simulink model "Australian14gen_inertia"  (R2017b)
settings: Solver=ode23tb  StartTime=0.0  StopTime=50  FixedStep=1e-3  RelTol=1e-3  AbsTol=1e-3  EnableMultiTasking=on
PreLoadFcn:
  | dataaustralian14gen
values from neighbouring files (symbols this model uses):
  alpha = -sys.follin.opt.alpha*1e8    [main_following.m]    (also in optimgains.mat = [-2447350365.29 -12566370614.4 -12566370614.4 -11730281347.7)
  bus_v = [ 101	15 ... (first row only)    [dataaustralian14gen.m]
  comp = [ 1	211	0	0 ... (first row only)    [dataaustralian14gen.m]
  dist = sys.follin.dist    [main_following.m]    (also in main_forming.m = sys.formin.dist)
  Exc = [ 101	0	 200	0.1	    13.25  2.5	 0	0       0       0       0       0 ... (first row only)    [dataaustralian14gen.m]
  FH = 13    [dataaustralian14gen.m]
  FI = 1    [dataaustralian14gen.m]
  FL = .1    (= 0.1)    [dataaustralian14gen.m]
  G_data = [ 101	333.3	15	3.6	0.14	1.1	0.65	0.25	8.5     0.25	0.05	0       0       0.25	0.2 	0 ... (first row only)    [dataaustralian14gen.m]
  KH = 120    [dataaustralian14gen.m]
  KI = 10    [dataaustralian14gen.m]
  KL = 10    [dataaustralian14gen.m]
  Kvsc = [-4.89904313526 -21.043852985 -7.4754770322 -20.8245159401 -7.65455531538 -20.65157337 -7.20128124012 -20.8334958357 -6.74777960012 -20.6206111903 -7.78863485578 -20.7555924998 ... (30 elements, 2x15)]    [optimgains.mat]
  line = [ 102	217	0.0084	0.0667	0.817	330	1 ... (first row only)    [dataaustralian14gen.m]
  load_mag = load_case4    [dataaustralian14gen.m]
  p = p_case4    [dataaustralian14gen.m]
  Pinit = zeros(15,1)    [dataaustralian14gen.m]
  PLL_Ki = 2/500    (= 0.004)    [dataaustralian14gen.m]
  PLL_Kp = 2/500    (= 0.004)    [dataaustralian14gen.m]
  PSSMODEL = 1    [dataaustralian14gen.m]
  trans = [ 1	101	102	15	330	333.3	12	12 ... (first row only)    [dataaustralian14gen.m]
undefined symbols (not defined in the file or in its folder): D1, Delta, sys, thetavsc0, Vbase
libraries: powerlib x388, Library x60, powerlib_meascontrol x15, sps_avr x10, powerlib_extras x4
(part 1 of 5)
Description:
  | SimPowerSystem model of the Simplified 14-Generator model
  | of the SE Australian Power System developed by Mike Gibbard & David Vowles,
  | School of Electrical & Electronic Engineering, The university of Adelaide, south australia)
  | 
  | SimPowerSystems model and validations by Ali Moeini and Innocent Kamwa,
  | IREQ, Hydro-Québec, Canada
settings Model: Creator=IREQ  LastModifiedBy=dominic
settings DataIOCC: LimitDataPoints=on  SaveFormat=Array
settings OptimizationCC: ExpressionDepthLimit=2147483647  LifeSpan=inf
settings DebuggingCC: UnderspecifiedInitializationDetection=Classic  MergeDetectMultiDrivingBlocksExec=none  IgnoredZcDiagnostic=none  SolverPrmCheckMsg=warning  UnconnectedInputMsg=none  UnconnectedOutputMsg=none  UnconnectedLineMsg=none  StateNameClashWarn=warning  SFUnexpectedBacktrackingDiag=warning  SFNoUnconditionalDefaultTransitionDiag=warning  SFExecutionAtInitializationDiag=none
settings HardwareCC: ProdBitPerPointer=32  ProdBitPerSizeT=32  ProdBitPerPtrDiffT=32  ProdLargestAtomicFloat=None  ProdIntDivRoundTo=Undefined  ProdEndianess=Unspecified  ProdWordSize=32  ProdHWDeviceType=32-bit Generic
settings ModelReferenceCC: PropagateSignalLabelsOutOfModel=off
settings CodeAppCC: StateflowObjectComments=on
settings GRTTargetCC: TargetLangStandard=C89/C90 (ANSI)  GeneratePreprocessorConditionals=Disable all
settings ConfigComp: CovMetricSettings=dw  CovHtmlReporting=on  CovSaveCumulativeToWorkspaceVar=on  CovSaveSingleToWorkspaceVar=on  CovExternalEMLEnable=off  CovSFcnEnable=off
settings SimscapeCC: SimscapeNormalizeSystem=off

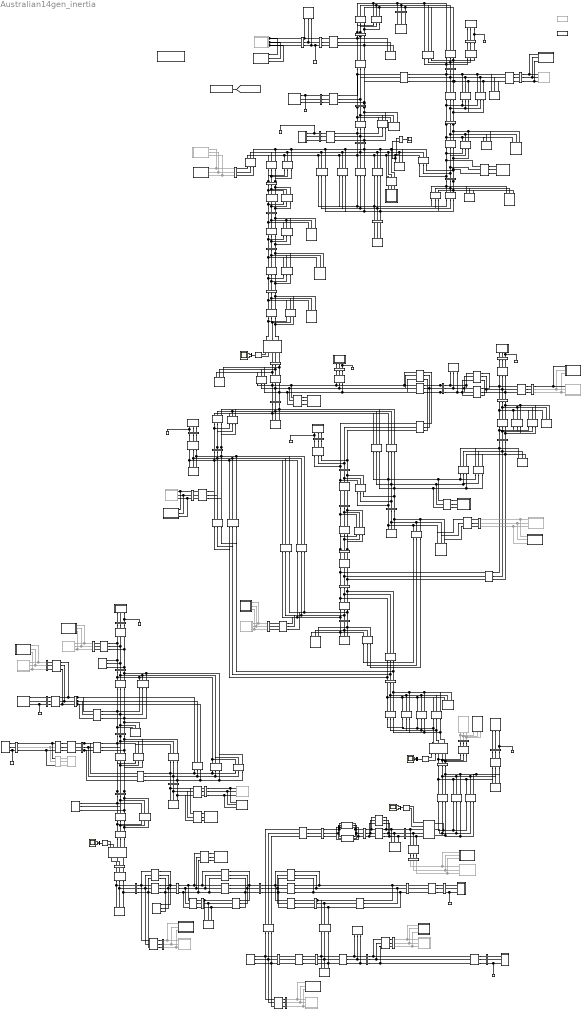
== system Australian14gen_inertia ==
  1 : powerlib/Elements/Three-Phase Series RLC Branch  LConnTagsString=A|B|C  RConnTagsString=A|B|C  BranchType=C  Resistance=0  Inductance=0  Capacitance=1/(0.0337)/(2*pi*50)*(330^2/100)  Measurements=None
  2 : powerlib/Elements/Three-Phase Series RLC Branch  LConnTagsString=A|B|C  RConnTagsString=A|B|C  BranchType=C  Resistance=0  Inductance=0  Capacitance=1/(0.0337)/(2*pi*50)*(330^2/100)  Measurements=None
  3-Phase Active & Reactive Power (Phasor Type){1..4} (4 alike) : powerlib_extras/Phasor Library/3-Phase Active & Reactive Power (Phasor Type)
  3-Phase Dynamic Load3 : powerlib/Elements/Three-Phase Dynamic Load  NominalVoltage=[ 15e3 50 ]  ActiveReactivePowers=[-5.4e+08 -4.56e+06]  PositiveSequence=[0.999196 -2.87767]  ExternalControl=off  NpNq="[0  0]"  TimeConstants=[0 0 0 0]  MinimumVoltage=0.01  Tfilter=1e-1  LoadFlowParameters=[4 50000000 0 0 25000000]
      settings: SourceProductName=Simscape Power Systems  SourceProductBaseCode=PS
  3-Phase Dynamic Load4 : powerlib/Elements/Three-Phase Dynamic Load  NominalVoltage=[ 15e3 50 ]  ActiveReactivePowers=[-1100 -2.11758e-14]  PositiveSequence=[1.08335 6.60259]  ExternalControl=off  NpNq="[0  0]"  TimeConstants=[0 0 0 0]  MinimumVoltage=0.01  Tfilter=1e-1  LoadFlowParameters=[4 50000000 0 0 25000000]
      settings: SourceProductName=Simscape Power Systems  SourceProductBaseCode=PS
  B101 : powerlib/Measurements/Three-Phase V-I Measurement  VoltageMeasurement=phase-to-phase  SetLabelV=on  LabelV=Vabc_B101  Vpu=off  VpuLL=off  CurrentMeasurement=no  SetLabelI=on  LabelI=Iabc_B101  Ipu=off  Pbase=100e6  Vbase=bus_v(1,2)*e3  OutputType=Complex  PhasorSimulation=on  PSBequivalent=0
  B102 : powerlib/Measurements/Three-Phase V-I Measurement  VoltageMeasurement=phase-to-ground  SetLabelV=on  LabelV=Vabc_B102  Vpu=off  VpuLL=off  CurrentMeasurement=yes  SetLabelI=on  LabelI=Iabc_B102  Ipu=off  Pbase=100e6  Vbase=bus_v(2,2)*e3  OutputType=Complex  PhasorSimulation=on  PSBequivalent=0
  B102_vi : powerlib/Measurements/Three-Phase V-I Measurement  VoltageMeasurement=phase-to-phase  SetLabelV=on  LabelV=Vabc_B102_vi  Vpu=off  VpuLL=off  CurrentMeasurement=no  SetLabelI=on  LabelI=Iabc_B101  Ipu=off  Pbase=100e6  Vbase=bus_v(1,2)*e3  OutputType=Complex  PhasorSimulation=on  PSBequivalent=0
  B201 : powerlib/Measurements/Three-Phase V-I Measurement  VoltageMeasurement=phase-to-phase  SetLabelV=on  LabelV=Vabc_B201  Vpu=off  VpuLL=off  CurrentMeasurement=no  SetLabelI=on  LabelI=Iabc_B201  Ipu=off  Pbase=100e6  Vbase=bus_v(3,2)*e3  OutputType=Complex  PhasorSimulation=on  PSBequivalent=0
  B202 : powerlib/Measurements/Three-Phase V-I Measurement  VoltageMeasurement=phase-to-phase  SetLabelV=on  LabelV=Vabc_B202  Vpu=off  VpuLL=off  CurrentMeasurement=no  SetLabelI=on  LabelI=Iabc_B202  Ipu=off  Pbase=100e6  Vbase=bus_v(4,2)*e3  OutputType=Complex  PhasorSimulation=on  PSBequivalent=0
  B203 : powerlib/Measurements/Three-Phase V-I Measurement  VoltageMeasurement=phase-to-phase  SetLabelV=on  LabelV=Vabc_B203  Vpu=off  VpuLL=off  CurrentMeasurement=no  SetLabelI=on  LabelI=Iabc_B203  Ipu=off  Pbase=100e6  Vbase=bus_v(5,2)*e3  OutputType=Complex  PhasorSimulation=on  PSBequivalent=0
  B204 : powerlib/Measurements/Three-Phase V-I Measurement  VoltageMeasurement=phase-to-phase  SetLabelV=on  LabelV=Vabc_B204  Vpu=off  VpuLL=off  CurrentMeasurement=no  SetLabelI=on  LabelI=Iabc_B204  Ipu=off  Pbase=100e6  Vbase=bus_v(6,2)*e3  OutputType=Complex  PhasorSimulation=on  PSBequivalent=0
  B205 : powerlib/Measurements/Three-Phase V-I Measurement  VoltageMeasurement=phase-to-ground  SetLabelV=on  LabelV=Vabc_B205  Vpu=off  VpuLL=off  CurrentMeasurement=yes  SetLabelI=on  LabelI=Iabc_B205  Ipu=off  Pbase=100e6  Vbase=bus_v(7,2)*e3  OutputType=Complex  PhasorSimulation=on  PSBequivalent=0
  B206 : powerlib/Measurements/Three-Phase V-I Measurement  VoltageMeasurement=phase-to-ground  SetLabelV=on  LabelV=Vabc_B206  Vpu=off  VpuLL=off  CurrentMeasurement=yes  SetLabelI=on  LabelI=Iabc_B206  Ipu=off  Pbase=100e6  Vbase=bus_v(8,2)*e3  OutputType=Complex  PhasorSimulation=on  PSBequivalent=0
  B207 : powerlib/Measurements/Three-Phase V-I Measurement  VoltageMeasurement=phase-to-ground  SetLabelV=on  LabelV=Vabc_B207  Vpu=off  VpuLL=off  CurrentMeasurement=yes  SetLabelI=on  LabelI=Iabc_B207  Ipu=off  Pbase=100e6  Vbase=138e3  OutputType=Complex  PhasorSimulation=on  PSBequivalent=0
  B208 : powerlib/Measurements/Three-Phase V-I Measurement  VoltageMeasurement=phase-to-ground  SetLabelV=on  LabelV=Vabc_B208  Vpu=off  VpuLL=off  CurrentMeasurement=yes  SetLabelI=on  LabelI=Iabc_B208  Ipu=off  Pbase=100e6  Vbase=138e3  OutputType=Complex  PhasorSimulation=on  PSBequivalent=0
  B208_vi : powerlib/Measurements/Three-Phase V-I Measurement  VoltageMeasurement=phase-to-phase  SetLabelV=on  LabelV=Vabc_B208_vi  Vpu=off  VpuLL=off  CurrentMeasurement=no  SetLabelI=on  LabelI=Iabc_B203  Ipu=off  Pbase=100e6  Vbase=bus_v(5,2)*e3  OutputType=Complex  PhasorSimulation=on  PSBequivalent=0
  B209 : powerlib/Measurements/Three-Phase V-I Measurement  VoltageMeasurement=phase-to-ground  SetLabelV=on  LabelV=Vabc_B209  Vpu=off  VpuLL=off  CurrentMeasurement=yes  SetLabelI=on  LabelI=Iabc_B209  Ipu=off  Pbase=100e6  Vbase=138e3  OutputType=Complex  PhasorSimulation=on  PSBequivalent=0
  B210 : powerlib/Measurements/Three-Phase V-I Measurement  VoltageMeasurement=phase-to-ground  SetLabelV=on  LabelV=Vabc_B210  Vpu=off  VpuLL=off  CurrentMeasurement=yes  SetLabelI=on  LabelI=Iabc_B210  Ipu=off  Pbase=100e6  Vbase=138e3  OutputType=Complex  PhasorSimulation=on  PSBequivalent=0
  B211 : powerlib/Measurements/Three-Phase V-I Measurement  VoltageMeasurement=phase-to-ground  SetLabelV=on  LabelV=Vabc_B211  Vpu=off  VpuLL=off  CurrentMeasurement=yes  SetLabelI=on  LabelI=Iabc_B211  Ipu=off  Pbase=100e6  Vbase=138e3  OutputType=Complex  PhasorSimulation=on  PSBequivalent=0
  B212 : powerlib/Measurements/Three-Phase V-I Measurement  VoltageMeasurement=phase-to-ground  SetLabelV=on  LabelV=Vabc_B212  Vpu=off  VpuLL=off  CurrentMeasurement=yes  SetLabelI=on  LabelI=Iabc_B212  Ipu=off  Pbase=100e6  Vbase=138e3  OutputType=Complex  PhasorSimulation=on  PSBequivalent=0
  B212_vi : powerlib/Measurements/Three-Phase V-I Measurement  VoltageMeasurement=phase-to-phase  SetLabelV=on  LabelV=Vabc_B212_vi  Vpu=off  VpuLL=off  CurrentMeasurement=no  SetLabelI=on  LabelI=Iabc_B203  Ipu=off  Pbase=100e6  Vbase=bus_v(5,2)*e3  OutputType=Complex  PhasorSimulation=on  PSBequivalent=0
  B213 : powerlib/Measurements/Three-Phase V-I Measurement  VoltageMeasurement=phase-to-ground  SetLabelV=on  LabelV=Vabc_B213  Vpu=off  VpuLL=off  CurrentMeasurement=yes  SetLabelI=on  LabelI=Iabc_B213  Ipu=off  Pbase=100e6  Vbase=138e3  OutputType=Complex  PhasorSimulation=on  PSBequivalent=0
  B214 : powerlib/Measurements/Three-Phase V-I Measurement  VoltageMeasurement=phase-to-ground  SetLabelV=on  LabelV=Vabc_B214  Vpu=off  VpuLL=off  CurrentMeasurement=yes  SetLabelI=on  LabelI=Iabc_B214  Ipu=off  Pbase=100e6  Vbase=138e3  OutputType=Complex  PhasorSimulation=on  PSBequivalent=0
  B215 : powerlib/Measurements/Three-Phase V-I Measurement  VoltageMeasurement=phase-to-ground  SetLabelV=on  LabelV=Vabc_B215  Vpu=off  VpuLL=off  CurrentMeasurement=yes  SetLabelI=on  LabelI=Iabc_B215  Ipu=off  Pbase=100e6  Vbase=138e3  OutputType=Complex  PhasorSimulation=on  PSBequivalent=0
  B215_vi : powerlib/Measurements/Three-Phase V-I Measurement  VoltageMeasurement=phase-to-phase  SetLabelV=on  LabelV=Vabc_B215_vi  Vpu=off  VpuLL=off  CurrentMeasurement=no  SetLabelI=on  LabelI=Iabc_B215  Ipu=off  Pbase=100e6  Vbase=138e3  OutputType=Complex  PhasorSimulation=on  PSBequivalent=0
  B216 : powerlib/Measurements/Three-Phase V-I Measurement  VoltageMeasurement=phase-to-ground  SetLabelV=on  LabelV=Vabc_B216  Vpu=off  VpuLL=off  CurrentMeasurement=yes  SetLabelI=on  LabelI=Iabc_B216  Ipu=off  Pbase=100e6  Vbase=138e3  OutputType=Complex  PhasorSimulation=on  PSBequivalent=0
  B216_vi : powerlib/Measurements/Three-Phase V-I Measurement  VoltageMeasurement=phase-to-phase  SetLabelV=on  LabelV=Vabc_B216_vi  Vpu=off  VpuLL=off  CurrentMeasurement=no  SetLabelI=off  LabelI=Iabc_B216  Ipu=off  Pbase=100e6  Vbase=138e3  OutputType=Complex  PhasorSimulation=on  PSBequivalent=0
  B217 : powerlib/Measurements/Three-Phase V-I Measurement  VoltageMeasurement=phase-to-ground  SetLabelV=on  LabelV=Vabc_B217  Vpu=off  VpuLL=off  CurrentMeasurement=yes  SetLabelI=on  LabelI=Iabc_B217  Ipu=off  Pbase=100e6  Vbase=138e3  OutputType=Complex  PhasorSimulation=on  PSBequivalent=0
  B301 : powerlib/Measurements/Three-Phase V-I Measurement  VoltageMeasurement=phase-to-phase  SetLabelV=on  LabelV=Vabc_B301  Vpu=off  VpuLL=off  CurrentMeasurement=no  SetLabelI=on  LabelI=Iabc_B301  Ipu=off  Pbase=100e6  Vbase=138e3  OutputType=Complex  PhasorSimulation=on  PSBequivalent=0
  B302 : powerlib/Measurements/Three-Phase V-I Measurement  VoltageMeasurement=phase-to-phase  SetLabelV=on  LabelV=Vabc_B302  Vpu=off  VpuLL=off  CurrentMeasurement=no  SetLabelI=on  LabelI=Iabc_B302  Ipu=off  Pbase=100e6  Vbase=138e3  OutputType=Complex  PhasorSimulation=on  PSBequivalent=0
  B303 : powerlib/Measurements/Three-Phase V-I Measurement  VoltageMeasurement=phase-to-ground  SetLabelV=on  LabelV=Vabc_B303  Vpu=off  VpuLL=off  CurrentMeasurement=yes  SetLabelI=on  LabelI=Iabc_B303  Ipu=off  Pbase=100e6  Vbase=138e3  OutputType=Complex  PhasorSimulation=on  PSBequivalent=0
  B304 : powerlib/Measurements/Three-Phase V-I Measurement  VoltageMeasurement=phase-to-ground  SetLabelV=on  LabelV=Vabc_B304  Vpu=off  VpuLL=off  CurrentMeasurement=yes  SetLabelI=on  LabelI=Iabc_B304  Ipu=off  Pbase=100e6  Vbase=138e3  OutputType=Complex  PhasorSimulation=on  PSBequivalent=0
  B305 : powerlib/Measurements/Three-Phase V-I Measurement  VoltageMeasurement=phase-to-ground  SetLabelV=on  LabelV=Vabc_B305  Vpu=off  VpuLL=off  CurrentMeasurement=yes  SetLabelI=on  LabelI=Iabc_B305  Ipu=off  Pbase=100e6  Vbase=138e3  OutputType=Complex  PhasorSimulation=on  PSBequivalent=0
  B306 : powerlib/Measurements/Three-Phase V-I Measurement  VoltageMeasurement=phase-to-ground  SetLabelV=on  LabelV=Vabc_B306  Vpu=off  VpuLL=off  CurrentMeasurement=yes  SetLabelI=on  LabelI=Iabc_B306  Ipu=off  Pbase=100e6  Vbase=138e3  OutputType=Complex  PhasorSimulation=on  PSBequivalent=0
  B307 : powerlib/Measurements/Three-Phase V-I Measurement  VoltageMeasurement=phase-to-ground  SetLabelV=on  LabelV=Vabc_B307  Vpu=off  VpuLL=off  CurrentMeasurement=yes  SetLabelI=on  LabelI=Iabc_B307  Ipu=off  Pbase=100e6  Vbase=138e3  OutputType=Complex  PhasorSimulation=on  PSBequivalent=0
  B308 : powerlib/Measurements/Three-Phase V-I Measurement  VoltageMeasurement=phase-to-ground  SetLabelV=on  LabelV=Vabc_B308  Vpu=off  VpuLL=off  CurrentMeasurement=yes  SetLabelI=on  LabelI=Iabc_B308  Ipu=off  Pbase=100e6  Vbase=138e3  OutputType=Complex  PhasorSimulation=on  PSBequivalent=0
  B308_vi : powerlib/Measurements/Three-Phase V-I Measurement  VoltageMeasurement=phase-to-phase  SetLabelV=on  LabelV=Vabc_B308_vi  Vpu=off  VpuLL=off  CurrentMeasurement=no  SetLabelI=on  LabelI=Iabc_B301  Ipu=off  Pbase=100e6  Vbase=138e3  OutputType=Complex  PhasorSimulation=on  PSBequivalent=0
  B309 : powerlib/Measurements/Three-Phase V-I Measurement  VoltageMeasurement=phase-to-ground  SetLabelV=on  LabelV=Vabc_B309  Vpu=off  VpuLL=off  CurrentMeasurement=yes  SetLabelI=on  LabelI=Iabc_B309  Ipu=off  Pbase=100e6  Vbase=138e3  OutputType=Complex  PhasorSimulation=on  PSBequivalent=0
  B309_vi : powerlib/Measurements/Three-Phase V-I Measurement  VoltageMeasurement=phase-to-phase  SetLabelV=on  LabelV=Vabc_B309_vi  Vpu=off  VpuLL=off  CurrentMeasurement=no  SetLabelI=off  LabelI=Iabc_B309  Ipu=off  Pbase=100e6  Vbase=138e3  OutputType=Complex  PhasorSimulation=on  PSBequivalent=0
  B310 : powerlib/Measurements/Three-Phase V-I Measurement  VoltageMeasurement=phase-to-ground  SetLabelV=on  LabelV=Vabc_B310  Vpu=off  VpuLL=off  CurrentMeasurement=yes  SetLabelI=on  LabelI=Iabc_B310  Ipu=off  Pbase=100e6  Vbase=138e3  OutputType=Complex  PhasorSimulation=on  PSBequivalent=0
  B311 : powerlib/Measurements/Three-Phase V-I Measurement  VoltageMeasurement=phase-to-ground  SetLabelV=on  LabelV=Vabc_B311  Vpu=off  VpuLL=off  CurrentMeasurement=yes  SetLabelI=on  LabelI=Iabc_B311  Ipu=off  Pbase=100e6  Vbase=138e3  OutputType=Complex  PhasorSimulation=on  PSBequivalent=0
  B312 : powerlib/Measurements/Three-Phase V-I Measurement  VoltageMeasurement=phase-to-ground  SetLabelV=on  LabelV=Vabc_B312  Vpu=off  VpuLL=off  CurrentMeasurement=yes  SetLabelI=on  LabelI=Iabc_B312  Ipu=off  Pbase=100e6  Vbase=138e3  OutputType=Complex  PhasorSimulation=on  PSBequivalent=0
  B312_vi : powerlib/Measurements/Three-Phase V-I Measurement  VoltageMeasurement=phase-to-phase  SetLabelV=on  LabelV=Vabc_B312_vi  Vpu=off  VpuLL=off  CurrentMeasurement=no  SetLabelI=off  LabelI=Iabc_B312_vi  Ipu=off  Pbase=100e6  Vbase=138e3  OutputType=Complex  PhasorSimulation=on  PSBequivalent=0
  B313 : powerlib/Measurements/Three-Phase V-I Measurement  VoltageMeasurement=phase-to-ground  SetLabelV=on  LabelV=Vabc_B313  Vpu=off  VpuLL=off  CurrentMeasurement=yes  SetLabelI=on  LabelI=Iabc_B313  Ipu=off  Pbase=100e6  Vbase=138e3  OutputType=Complex  PhasorSimulation=on  PSBequivalent=0
  B314 : powerlib/Measurements/Three-Phase V-I Measurement  VoltageMeasurement=phase-to-ground  SetLabelV=on  LabelV=Vabc_B314  Vpu=off  VpuLL=off  CurrentMeasurement=yes  SetLabelI=on  LabelI=Iabc_B314  Ipu=off  Pbase=100e6  Vbase=138e3  OutputType=Complex  PhasorSimulation=on  PSBequivalent=0
  B314_vi : powerlib/Measurements/Three-Phase V-I Measurement  VoltageMeasurement=phase-to-phase  SetLabelV=on  LabelV=Vabc_B314_vi  Vpu=off  VpuLL=off  CurrentMeasurement=no  SetLabelI=off  LabelI=Iabc_B314_vi  Ipu=off  Pbase=100e6  Vbase=138e3  OutputType=Complex  PhasorSimulation=on  PSBequivalent=0
  B315 : powerlib/Measurements/Three-Phase V-I Measurement  VoltageMeasurement=phase-to-ground  SetLabelV=on  LabelV=Vabc_B315  Vpu=off  VpuLL=off  CurrentMeasurement=yes  SetLabelI=on  LabelI=Iabc_B315  Ipu=off  Pbase=100e6  Vbase=138e3  OutputType=Complex  PhasorSimulation=on  PSBequivalent=0
  B401 : powerlib/Measurements/Three-Phase V-I Measurement  VoltageMeasurement=phase-to-phase  SetLabelV=on  LabelV=Vabc_B401  Vpu=off  VpuLL=off  CurrentMeasurement=no  SetLabelI=on  LabelI=Iabc_B401  Ipu=off  Pbase=100e6  Vbase=138e3  OutputType=Complex  PhasorSimulation=on  PSBequivalent=0
  B402 : powerlib/Measurements/Three-Phase V-I Measurement  VoltageMeasurement=phase-to-phase  SetLabelV=on  LabelV=Vabc_B402  Vpu=off  VpuLL=off  CurrentMeasurement=no  SetLabelI=off  LabelI=Iabc_B402  Ipu=off  Pbase=100e6  Vbase=138e3  OutputType=Complex  PhasorSimulation=on  PSBequivalent=0
  B403 : powerlib/Measurements/Three-Phase V-I Measurement  VoltageMeasurement=phase-to-phase  SetLabelV=on  LabelV=Vabc_B403  Vpu=off  VpuLL=off  CurrentMeasurement=no  SetLabelI=on  LabelI=Iabc_B403  Ipu=off  Pbase=100e6  Vbase=138e3  OutputType=Complex  PhasorSimulation=on  PSBequivalent=0
  B403_vi : powerlib/Measurements/Three-Phase V-I Measurement  VoltageMeasurement=phase-to-phase  SetLabelV=on  LabelV=Vabc_B403_vi  Vpu=off  VpuLL=off  CurrentMeasurement=no  SetLabelI=on  LabelI=Iabc_B403  Ipu=off  Pbase=100e6  Vbase=138e3  OutputType=Complex  PhasorSimulation=on  PSBequivalent=0
  B404 : powerlib/Measurements/Three-Phase V-I Measurement  VoltageMeasurement=phase-to-phase  SetLabelV=on  LabelV=Vabc_B404  Vpu=off  VpuLL=off  CurrentMeasurement=no  SetLabelI=on  LabelI=Iabc_B404  Ipu=off  Pbase=100e6  Vbase=138e3  OutputType=Complex  PhasorSimulation=on  PSBequivalent=0
  B405 : powerlib/Measurements/Three-Phase V-I Measurement  VoltageMeasurement=phase-to-ground  SetLabelV=on  LabelV=Vabc_B405  Vpu=off  VpuLL=off  CurrentMeasurement=yes  SetLabelI=on  LabelI=Iabc_B405  Ipu=off  Pbase=100e6  Vbase=138e3  OutputType=Complex  PhasorSimulation=on  PSBequivalent=0
  B405_vi : powerlib/Measurements/Three-Phase V-I Measurement  VoltageMeasurement=phase-to-phase  SetLabelV=on  LabelV=Vabc_B405_vi  Vpu=off  VpuLL=off  CurrentMeasurement=no  SetLabelI=on  LabelI=Iabc_B404  Ipu=off  Pbase=100e6  Vbase=138e3  OutputType=Complex  PhasorSimulation=on  PSBequivalent=0
  B406 : powerlib/Measurements/Three-Phase V-I Measurement  VoltageMeasurement=phase-to-ground  SetLabelV=on  LabelV=Vabc_B406  Vpu=off  VpuLL=off  CurrentMeasurement=yes  SetLabelI=on  LabelI=Iabc_B406  Ipu=off  Pbase=100e6  Vbase=138e3  OutputType=Complex  PhasorSimulation=on  PSBequivalent=0
  B407 : powerlib/Measurements/Three-Phase V-I Measurement  VoltageMeasurement=phase-to-ground  SetLabelV=on  LabelV=Vabc_B407  Vpu=off  VpuLL=off  CurrentMeasurement=yes  SetLabelI=on  LabelI=Iabc_B407  Ipu=off  Pbase=100e6  Vbase=138e3  OutputType=Complex  PhasorSimulation=on  PSBequivalent=0
  B408 : powerlib/Measurements/Three-Phase V-I Measurement  VoltageMeasurement=phase-to-ground  SetLabelV=on  LabelV=Vabc_B408  Vpu=off  VpuLL=off  CurrentMeasurement=yes  SetLabelI=on  LabelI=Iabc_B408  Ipu=off  Pbase=100e6  Vbase=138e3  OutputType=Complex  PhasorSimulation=on  PSBequivalent=0
  B409 : powerlib/Measurements/Three-Phase V-I Measurement  VoltageMeasurement=phase-to-ground  SetLabelV=on  LabelV=Vabc_B409  Vpu=off  VpuLL=off  CurrentMeasurement=yes  SetLabelI=on  LabelI=Iabc_B409  Ipu=off  Pbase=100e6  Vbase=138e3  OutputType=Complex  PhasorSimulation=on  PSBequivalent=0
  B410 : powerlib/Measurements/Three-Phase V-I Measurement  VoltageMeasurement=phase-to-ground  SetLabelV=on  LabelV=Vabc_B410  Vpu=off  VpuLL=off  CurrentMeasurement=no  SetLabelI=on  LabelI=Iabc_B410  Ipu=off  Pbase=100e6  Vbase=138e3  OutputType=Magnitude  PhasorSimulation=on  PSBequivalent=0
  B410_vi : powerlib/Measurements/Three-Phase V-I Measurement  VoltageMeasurement=phase-to-phase  SetLabelV=on  LabelV=Vabc_B410_vi  Vpu=off  VpuLL=off  CurrentMeasurement=no  SetLabelI=on  LabelI=Iabc_B401  Ipu=off  Pbase=100e6  Vbase=138e3  OutputType=Complex  PhasorSimulation=on  PSBequivalent=0
  B411 : powerlib/Measurements/Three-Phase V-I Measurement  VoltageMeasurement=phase-to-ground  SetLabelV=on  LabelV=Vabc_B411  Vpu=off  VpuLL=off  CurrentMeasurement=yes  SetLabelI=on  LabelI=Iabc_B411  Ipu=off  Pbase=100e6  Vbase=138e3  OutputType=Complex  PhasorSimulation=on  PSBequivalent=0
  B412 : powerlib/Measurements/Three-Phase V-I Measurement  VoltageMeasurement=phase-to-ground  SetLabelV=on  LabelV=Vabc_B412  Vpu=off  VpuLL=off  CurrentMeasurement=yes  SetLabelI=on  LabelI=Iabc_B412  Ipu=off  Pbase=100e6  Vbase=138e3  OutputType=Complex  PhasorSimulation=on  PSBequivalent=0
  B413 : powerlib/Measurements/Three-Phase V-I Measurement  VoltageMeasurement=phase-to-ground  SetLabelV=on  LabelV=Vabc_B413  Vpu=off  VpuLL=off  CurrentMeasurement=yes  SetLabelI=on  LabelI=Iabc_B413  Ipu=off  Pbase=100e6  Vbase=138e3  OutputType=Complex  PhasorSimulation=on  PSBequivalent=0
  B414 : powerlib/Measurements/Three-Phase V-I Measurement  VoltageMeasurement=phase-to-ground  SetLabelV=on  LabelV=Vabc_B414  Vpu=off  VpuLL=off  CurrentMeasurement=yes  SetLabelI=on  LabelI=Iabc_B414  Ipu=off  Pbase=100e6  Vbase=138e3  OutputType=Complex  PhasorSimulation=on  PSBequivalent=0
  B415 : powerlib/Measurements/Three-Phase V-I Measurement  VoltageMeasurement=phase-to-ground  SetLabelV=on  LabelV=Vabc_B415  Vpu=off  VpuLL=off  CurrentMeasurement=yes  SetLabelI=on  LabelI=Iabc_B415  Ipu=off  Pbase=100e6  Vbase=138e3  OutputType=Complex  PhasorSimulation=on  PSBequivalent=0
  B416 : powerlib/Measurements/Three-Phase V-I Measurement  VoltageMeasurement=phase-to-ground  SetLabelV=on  LabelV=Vabc_B416  Vpu=off  VpuLL=off  CurrentMeasurement=yes  SetLabelI=on  LabelI=Iabc_B416  Ipu=off  Pbase=100e6  Vbase=138e3  OutputType=Complex  PhasorSimulation=on  PSBequivalent=0
  B501 : powerlib/Measurements/Three-Phase V-I Measurement  VoltageMeasurement=phase-to-phase  SetLabelV=on  LabelV=Vabc_B501  Vpu=off  VpuLL=off  CurrentMeasurement=no  SetLabelI=on  LabelI=Iabc_B501  Ipu=off  Pbase=100e6  Vbase=138e3  OutputType=Complex  PhasorSimulation=on  PSBequivalent=0
  B502 : powerlib/Measurements/Three-Phase V-I Measurement  VoltageMeasurement=phase-to-phase  SetLabelV=on  LabelV=Vabc_B502  Vpu=off  VpuLL=off  CurrentMeasurement=no  SetLabelI=on  LabelI=Iabc_B502  Ipu=off  Pbase=100e6  Vbase=138e3  OutputType=Complex  PhasorSimulation=on  PSBequivalent=0
  B502_vi : powerlib/Measurements/Three-Phase V-I Measurement  VoltageMeasurement=phase-to-phase  SetLabelV=on  LabelV=Vabc_B502_vi  Vpu=off  VpuLL=off  CurrentMeasurement=no  SetLabelI=on  LabelI=Iabc_B502  Ipu=off  Pbase=100e6  Vbase=138e3  OutputType=Complex  PhasorSimulation=on  PSBequivalent=0
  B503 : powerlib/Measurements/Three-Phase V-I Measurement  VoltageMeasurement=phase-to-phase  SetLabelV=on  LabelV=Vabc_B503  Vpu=off  VpuLL=off  CurrentMeasurement=yes  SetLabelI=on  LabelI=Iabc_B503  Ipu=off  Pbase=100e6  Vbase=138e3  OutputType=Complex  PhasorSimulation=on  PSBequivalent=0
  B504 : powerlib/Measurements/Three-Phase V-I Measurement  VoltageMeasurement=phase-to-ground  SetLabelV=on  LabelV=Vabc_B504  Vpu=off  VpuLL=off  CurrentMeasurement=yes  SetLabelI=on  LabelI=Iabc_B504  Ipu=off  Pbase=100e6  Vbase=138e3  OutputType=Complex  PhasorSimulation=on  PSBequivalent=0
  B504_vi : powerlib/Measurements/Three-Phase V-I Measurement  VoltageMeasurement=phase-to-phase  SetLabelV=on  LabelV=Vabc_B504_vi  Vpu=off  VpuLL=off  CurrentMeasurement=no  SetLabelI=on  LabelI=Iabc_B502  Ipu=off  Pbase=100e6  Vbase=138e3  OutputType=Complex  PhasorSimulation=on  PSBequivalent=0
  B505 : powerlib/Measurements/Three-Phase V-I Measurement  VoltageMeasurement=phase-to-ground  SetLabelV=on  LabelV=Vabc_B505  Vpu=off  VpuLL=off  CurrentMeasurement=yes  SetLabelI=on  LabelI=Iabc_B505  Ipu=off  Pbase=100e6  Vbase=138e3  OutputType=Complex  PhasorSimulation=on  PSBequivalent=0
  B506 : powerlib/Measurements/Three-Phase V-I Measurement  VoltageMeasurement=phase-to-ground  SetLabelV=on  LabelV=Vabc_B506  Vpu=off  VpuLL=off  CurrentMeasurement=yes  SetLabelI=on  LabelI=Iabc_B506  Ipu=off  Pbase=100e6  Vbase=138e3  OutputType=Complex  PhasorSimulation=on  PSBequivalent=0
  B507 : powerlib/Measurements/Three-Phase V-I Measurement  VoltageMeasurement=phase-to-ground  SetLabelV=on  LabelV=Vabc_B507  Vpu=off  VpuLL=off  CurrentMeasurement=yes  SetLabelI=on  LabelI=Iabc_B507  Ipu=off  Pbase=100e6  Vbase=138e3  OutputType=Complex  PhasorSimulation=on  PSBequivalent=0
  B508 : powerlib/Measurements/Three-Phase V-I Measurement  VoltageMeasurement=phase-to-ground  SetLabelV=on  LabelV=Vabc_B508  Vpu=off  VpuLL=off  CurrentMeasurement=yes  SetLabelI=on  LabelI=Iabc_B508  Ipu=off  Pbase=100e6  Vbase=138e3  OutputType=Complex  PhasorSimulation=on  PSBequivalent=0
  B508_vi : powerlib/Measurements/Three-Phase V-I Measurement  VoltageMeasurement=phase-to-phase  SetLabelV=on  LabelV=Vabc_B508_vi  Vpu=off  VpuLL=off  CurrentMeasurement=no  SetLabelI=off  LabelI=Iabc_B503  Ipu=off  Pbase=100e6  Vbase=138e3  OutputType=Complex  PhasorSimulation=on  PSBequivalent=0
  B509 : powerlib/Measurements/Three-Phase V-I Measurement  VoltageMeasurement=phase-to-ground  SetLabelV=on  LabelV=Vabc_B3509  Vpu=off  VpuLL=off  CurrentMeasurement=yes  SetLabelI=on  LabelI=Iabc_B509  Ipu=off  Pbase=100e6  Vbase=138e3  OutputType=Complex  PhasorSimulation=on  PSBequivalent=0
  CPS402 : powerlib/Elements/Three-Phase Dynamic Load  NominalVoltage=[ 20e3 50 ]  ActiveReactivePowers=[-5.86e+08 1.015e+07]  PositiveSequence=[0.996609 19.5]  ExternalControl=off  NpNq="[0  0]"  TimeConstants=[0 0 0 0]  MinimumVoltage=0.01  Tfilter=1e-1  LoadFlowParameters=[4 50000000 0 0 25000000]
      settings: SourceProductName=Simscape Power Systems  SourceProductBaseCode=PS
  CPS403 : powerlib/Elements/Three-Phase Dynamic Load  NominalVoltage=[ 20e3 50 ]  ActiveReactivePowers=[-9.655e+08 -3.808e+07]  PositiveSequence=[0.997203 20.5817]  ExternalControl=off  NpNq="[0  0]"  TimeConstants=[0 0 0 0]  MinimumVoltage=0.01  Tfilter=1e-1  LoadFlowParameters=[4 50000000 0 0 25000000]
      settings: SourceProductName=Simscape Power Systems  SourceProductBaseCode=PS
  Comp2-212 : powerlib/Elements/Three-Phase Parallel RLC Load  LConnTagsString=A|B|C  Configuration=Y (grounded)  NominalVoltage=(330000)*1  Vabc=[1e3 1e3 1e3]  Vabcp=[1e3 1e3 1e3]  NominalFrequency=50  UnbalancedPower=off  ActivePower=0  InductivePower=comp(2,3)*1e6  CapacitivePower=comp(2,4)*1e6  Pabc=[10e3 9e3 11e3]  QLabc=[100 90 110]  QCabc=[100 90 110]  Pabcp=[10e3 9e3 11e3]  QLabcp=[100 90 110]  QCabcp=[100 90 110]  Measurements=None  LoadType=constant Z
  Comp3-216 : powerlib/Elements/Three-Phase Parallel RLC Load  LConnTagsString=A|B|C  Configuration=Y (grounded)  NominalVoltage=(330000)*1  Vabc=[1e3 1e3 1e3]  Vabcp=[1e3 1e3 1e3]  NominalFrequency=50  UnbalancedPower=off  ActivePower=0  InductivePower=comp(3,3)*1e6  CapacitivePower=comp(3,4)*1e6  Pabc=[10e3 9e3 11e3]  QLabc=[100 90 110]  QCabc=[100 90 110]  Pabcp=[10e3 9e3 11e3]  QLabcp=[100 90 110]  QCabcp=[100 90 110]  Measurements=None  LoadType=constant Z
  Comp4-409 : powerlib/Elements/Three-Phase Parallel RLC Load  LConnTagsString=A|B|C  Configuration=Y (grounded)  NominalVoltage=(275000)*1  Vabc=[1e3 1e3 1e3]  Vabcp=[1e3 1e3 1e3]  NominalFrequency=50  UnbalancedPower=off  ActivePower=0  InductivePower=comp(4,3)*1e6  CapacitivePower=comp(4,4)*1e6  Pabc=[10e3 9e3 11e3]  QLabc=[100 90 110]  QCabc=[100 90 110]  Pabcp=[10e3 9e3 11e3]  QLabcp=[100 90 110]  QCabcp=[100 90 110]  Measurements=None  LoadType=constant Z
  Comp5-411 : powerlib/Elements/Three-Phase Parallel RLC Load  LConnTagsString=A|B|C  Configuration=Y (grounded)  NominalVoltage=(275000)*1  Vabc=[1e3 1e3 1e3]  Vabcp=[1e3 1e3 1e3]  NominalFrequency=50  UnbalancedPower=off  ActivePower=0  InductivePower=comp(5,3)*1e6  CapacitivePower=comp(5,4)*1e6  Pabc=[10e3 9e3 11e3]  QLabc=[100 90 110]  QCabc=[100 90 110]  Pabcp=[10e3 9e3 11e3]  QLabcp=[100 90 110]  QCabcp=[100 90 110]  Measurements=None  LoadType=constant Z
  Comp6-414 : powerlib/Elements/Three-Phase Parallel RLC Load  LConnTagsString=A|B|C  Configuration=Y (grounded)  NominalVoltage=(330000)*1  Vabc=[1e3 1e3 1e3]  Vabcp=[1e3 1e3 1e3]  NominalFrequency=50  UnbalancedPower=off  ActivePower=0  InductivePower=comp(6,3)*1e6  CapacitivePower=comp(6,4)*1e6  Pabc=[10e3 9e3 11e3]  QLabc=[100 90 110]  QCabc=[100 90 110]  Pabcp=[10e3 9e3 11e3]  QLabcp=[100 90 110]  QCabcp=[100 90 110]  Measurements=None  LoadType=constant Z
  Comp7-415 : powerlib/Elements/Three-Phase Parallel RLC Load  LConnTagsString=A|B|C  Configuration=Y (grounded)  NominalVoltage=(330000)*1  Vabc=[1e3 1e3 1e3]  Vabcp=[1e3 1e3 1e3]  NominalFrequency=50  UnbalancedPower=off  ActivePower=0  InductivePower=comp(7,3)*1e6  CapacitivePower=comp(7,4)*1e6  Pabc=[10e3 9e3 11e3]  QLabc=[100 90 110]  QCabc=[100 90 110]  Pabcp=[10e3 9e3 11e3]  QLabcp=[100 90 110]  QCabcp=[100 90 110]  Measurements=None  LoadType=constant Z
  Comp8-416 : powerlib/Elements/Three-Phase Parallel RLC Load  LConnTagsString=A|B|C  Configuration=Y (grounded)  NominalVoltage=(330000)*1  Vabc=[1e3 1e3 1e3]  Vabcp=[1e3 1e3 1e3]  NominalFrequency=50  UnbalancedPower=off  ActivePower=0  InductivePower=comp(8,3)*1e6  CapacitivePower=comp(8,4)*1e6  Pabc=[10e3 9e3 11e3]  QLabc=[100 90 110]  QCabc=[100 90 110]  Pabcp=[10e3 9e3 11e3]  QLabcp=[100 90 110]  QCabcp=[100 90 110]  Measurements=None  LoadType=constant Z
  Demux{,1..3} (4 alike) : Demux  Outputs=2
  Dist206 : Subsystem
  Dist212 : Subsystem
  Dist307 : Subsystem
  Dist410 : Subsystem
  Dist411 : Subsystem
  Dist508 : Subsystem
  G201_BPS : Subsystem
  G202_EPS : Subsystem
  G203_VPS : Subsystem
  G204_MPS : Subsystem
  G301_LPS : Subsystem
  G302_YPS : Subsystem
  G401_TPS : Subsystem
  G404_GPS : Subsystem
  G501_NPS : Subsystem
  G503_PPS : Subsystem
  L-1-1 : powerlib/Elements/Three-Phase PI Section Line  LConnTagsString=a|b|c  RConnTagsString=A|B|C  Frequency=50  Resistances="[ line(1,3)  line(1,3)*3]"  Inductances="[ line(1,4)  line(1,4)*3]"  Capacitances="[ line(1,5)  line(1,5)/3]"  Length=1
      settings: SourceProductName=Simscape Power Systems
  L-1-2 : powerlib/Elements/Three-Phase PI Section Line  LConnTagsString=a|b|c  RConnTagsString=A|B|C  Frequency=50  Resistances="[ line(1,3)  line(1,3)*3]"  Inductances="[ line(1,4)  line(1,4)*3]"  Capacitances="[ line(1,5)  line(1,5)/3]"  Length=1
      settings: SourceProductName=Simscape Power Systems
  L-10-1 : powerlib/Elements/Three-Phase PI Section Line  LConnTagsString=a|b|c  RConnTagsString=A|B|C  Frequency=50  Resistances="[ line(10,3)  line(10,3)*3]"  Inductances="[ line(10,4)  line(10,4)*3]"  Capacitances="[ line(10,5)  line(10,5)/3]"  Length=1
      settings: SourceProductName=Simscape Power Systems
  L-10-2 : powerlib/Elements/Three-Phase PI Section Line  LConnTagsString=a|b|c  RConnTagsString=A|B|C  Frequency=50  Resistances="[ line(10,3)  line(10,3)*3]"  Inductances="[ line(10,4)  line(10,4)*3]"  Capacitances="[ line(10,5)  line(10,5)/3]"  Length=1
      settings: SourceProductName=Simscape Power Systems
  L-11 : powerlib/Elements/Three-Phase PI Section Line  LConnTagsString=a|b|c  RConnTagsString=A|B|C  Frequency=50  Resistances="[ line(11,3)  line(11,3)*3]"  Inductances="[ line(11,4)  line(11,4)*3]"  Capacitances="[ line(11,5)  line(11,5)/3]"  Length=1
      settings: SourceProductName=Simscape Power Systems
  L-12-1 : powerlib/Elements/Three-Phase PI Section Line  LConnTagsString=a|b|c  RConnTagsString=A|B|C  Frequency=50  Resistances="[ line(12,3)  line(12,3)*3]"  Inductances="[ line(12,4)  line(12,4)*3]"  Capacitances="[ line(12,5)  line(12,5)/3]"  Length=1
      settings: SourceProductName=Simscape Power Systems
  L-12-2 : powerlib/Elements/Three-Phase PI Section Line  LConnTagsString=a|b|c  RConnTagsString=A|B|C  Frequency=50  Resistances="[ line(12,3)  line(12,3)*3]"  Inductances="[ line(12,4)  line(12,4)*3]"  Capacitances="[ line(12,5)  line(12,5)/3]"  Length=1
      settings: SourceProductName=Simscape Power Systems
  L-12-3 : powerlib/Elements/Three-Phase PI Section Line  LConnTagsString=a|b|c  RConnTagsString=A|B|C  Frequency=50  Resistances="[ line(12,3)  line(12,3)*3]"  Inductances="[ line(12,4)  line(12,4)*3]"  Capacitances="[ line(12,5)  line(12,5)/3]"  Length=1
      settings: SourceProductName=Simscape Power Systems
  L-13 : powerlib/Elements/Three-Phase PI Section Line  LConnTagsString=a|b|c  RConnTagsString=A|B|C  Frequency=50  Resistances="[ line(13,3)  line(13,3)*3]"  Inductances="[ line(13,4)  line(13,4)*3]"  Capacitances="[ line(13,5)  line(13,5)/3]"  Length=1
      settings: SourceProductName=Simscape Power Systems
  L-14-1 : powerlib/Elements/Three-Phase PI Section Line  LConnTagsString=a|b|c  RConnTagsString=A|B|C  Frequency=50  Resistances="[ line(14,3)  line(14,3)*3]"  Inductances="[ line(14,4)  line(14,4)*3]"  Capacitances="[ line(14,5)  line(14,5)/3]"  Length=1
      settings: SourceProductName=Simscape Power Systems
  L-14-2 : powerlib/Elements/Three-Phase PI Section Line  LConnTagsString=a|b|c  RConnTagsString=A|B|C  Frequency=50  Resistances="[ line(14,3)  line(14,3)*3]"  Inductances="[ line(14,4)  line(14,4)*3]"  Capacitances="[ line(14,5)  line(14,5)/3]"  Length=1
      settings: SourceProductName=Simscape Power Systems
  L-15-1 : powerlib/Elements/Three-Phase PI Section Line  LConnTagsString=a|b|c  RConnTagsString=A|B|C  Frequency=50  Resistances="[ line(15,3)  line(15,3)*3]"  Inductances="[ line(15,4)  line(15,4)*3]"  Capacitances="[ line(15,5)  line(15,5)/3]"  Length=1
      settings: SourceProductName=Simscape Power Systems
  L-15-2 : powerlib/Elements/Three-Phase PI Section Line  LConnTagsString=a|b|c  RConnTagsString=A|B|C  Frequency=50  Resistances="[ line(15,3)  line(15,3)*3]"  Inductances="[ line(15,4)  line(15,4)*3]"  Capacitances="[ line(15,5)  line(15,5)/3]"  Length=1
      settings: SourceProductName=Simscape Power Systems
  L-16 : powerlib/Elements/Three-Phase PI Section Line  LConnTagsString=a|b|c  RConnTagsString=A|B|C  Frequency=50  Resistances="[ line(16,3)  line(16,3)*3]"  Inductances="[ line(16,4)  line(16,4)*3]"  Capacitances="[ line(16,5)  line(16,5)/3]"  Length=1
      settings: SourceProductName=Simscape Power Systems
  L-17 : powerlib/Elements/Three-Phase PI Section Line  LConnTagsString=a|b|c  RConnTagsString=A|B|C  Frequency=50  Resistances="[ line(17,3)  line(17,3)*3]"  Inductances="[ line(17,4)  line(17,4)*3]"  Capacitances="[ line(17,5)  line(17,5)/3]"  Length=1
      settings: SourceProductName=Simscape Power Systems
  L-18 : powerlib/Elements/Three-Phase PI Section Line  LConnTagsString=a|b|c  RConnTagsString=A|B|C  Frequency=50  Resistances="[ line(18,3)  line(18,3)*3]"  Inductances="[ line(18,4)  line(18,4)*3]"  Capacitances="[ line(18,5)  line(18,5)/3]"  Length=1
      settings: SourceProductName=Simscape Power Systems
  L-19 : powerlib/Elements/Three-Phase PI Section Line  LConnTagsString=a|b|c  RConnTagsString=A|B|C  Frequency=50  Resistances="[ line(19,3)  line(19,3)*3]"  Inductances="[ line(19,4)  line(19,4)*3]"  Capacitances="[ line(19,5)  line(19,5)/3]"  Length=1
      settings: SourceProductName=Simscape Power Systems
  L-2-1 : powerlib/Elements/Three-Phase PI Section Line  LConnTagsString=a|b|c  RConnTagsString=A|B|C  Frequency=50  Resistances="[ line(2,3)  line(2,3)*3]"  Inductances="[ line(2,4)  line(2,4)*3]"  Capacitances="[ line(2,5)  line(2,5)/3]"  Length=1
      settings: SourceProductName=Simscape Power Systems
  L-2-2 : powerlib/Elements/Three-Phase PI Section Line  LConnTagsString=a|b|c  RConnTagsString=A|B|C  Frequency=50  Resistances="[ line(2,3)  line(2,3)*3]"  Inductances="[ line(2,4)  line(2,4)*3]"  Capacitances="[ line(2,5)  line(2,5)/3]"  Length=1
      settings: SourceProductName=Simscape Power Systems
  L-20-1 : powerlib/Elements/Three-Phase PI Section Line  LConnTagsString=a|b|c  RConnTagsString=A|B|C  Frequency=50  Resistances="[ line(20,3)  line(20,3)*3]"  Inductances="[ line(20,4)  line(20,4)*3]"  Capacitances="[ line(20,5)  line(20,5)/3]"  Length=1
      settings: SourceProductName=Simscape Power Systems
  L-20-2 : powerlib/Elements/Three-Phase PI Section Line  LConnTagsString=a|b|c  RConnTagsString=A|B|C  Frequency=50  Resistances="[ line(20,3)  line(20,3)*3]"  Inductances="[ line(20,4)  line(20,4)*3]"  Capacitances="[ line(20,5)  line(20,5)/3]"  Length=1
      settings: SourceProductName=Simscape Power Systems
  L-21-1 : powerlib/Elements/Three-Phase PI Section Line  LConnTagsString=a|b|c  RConnTagsString=A|B|C  Frequency=50  Resistances="[ line(21,3)  line(21,3)*3]"  Inductances="[ line(21,4)  line(21,4)*3]"  Capacitances="[ line(21,5)  line(21,5)/3]"  Length=1
      settings: SourceProductName=Simscape Power Systems
  L-21-2 : powerlib/Elements/Three-Phase PI Section Line  LConnTagsString=a|b|c  RConnTagsString=A|B|C  Frequency=50  Resistances="[ line(21,3)  line(21,3)*3]"  Inductances="[ line(21,4)  line(21,4)*3]"  Capacitances="[ line(21,5)  line(21,5)/3]"  Length=1
      settings: SourceProductName=Simscape Power Systems
  L-22 : powerlib/Elements/Three-Phase PI Section Line  LConnTagsString=a|b|c  RConnTagsString=A|B|C  Frequency=50  Resistances="[ line(22,3)  line(22,3)*3]"  Inductances="[ line(22,4)  line(22,4)*3]"  Capacitances="[ line(22,5)  line(22,5)/3]"  Length=1
      settings: SourceProductName=Simscape Power Systems
  L-23 : powerlib/Elements/Three-Phase PI Section Line  LConnTagsString=a|b|c  RConnTagsString=A|B|C  Frequency=50  Resistances="[ line(23,3)  line(23,3)*3]"  Inductances="[ line(23,4)  line(23,4)*3]"  Capacitances="[ line(23,5)  line(23,5)/3]"  Length=1
      settings: SourceProductName=Simscape Power Systems
  L-24-1 : powerlib/Elements/Three-Phase PI Section Line  LConnTagsString=a|b|c  RConnTagsString=A|B|C  Frequency=50  Resistances="[ line(24,3)  line(24,3)*3]"  Inductances="[ line(24,4)  line(24,4)*3]"  Capacitances="[ line(24,5)  line(24,5)/3]"  Length=1
      settings: SourceProductName=Simscape Power Systems
  L-24-2 : powerlib/Elements/Three-Phase PI Section Line  LConnTagsString=a|b|c  RConnTagsString=A|B|C  Frequency=50  Resistances="[ line(24,3)  line(24,3)*3]"  Inductances="[ line(24,4)  line(24,4)*3]"  Capacitances="[ line(24,5)  line(24,5)/3]"  Length=1
      settings: SourceProductName=Simscape Power Systems
  L-25 : powerlib/Elements/Three-Phase PI Section Line  LConnTagsString=a|b|c  RConnTagsString=A|B|C  Frequency=50  Resistances="[ line(25,3)  line(25,3)*3]"  Inductances="[ line(25,4)  line(25,4)*3]"  Capacitances="[ line(25,5)  line(25,5)/3]"  Length=1
      settings: SourceProductName=Simscape Power Systems
  L-26 : powerlib/Elements/Three-Phase PI Section Line  LConnTagsString=a|b|c  RConnTagsString=A|B|C  Frequency=50  Resistances="[ line(26,3)  line(26,3)*3]"  Inductances="[ line(26,4)  line(26,4)*3]"  Capacitances="[ line(26,5)  line(26,5)/3]"  Length=1
      settings: SourceProductName=Simscape Power Systems
  L-27-1 : powerlib/Elements/Three-Phase PI Section Line  LConnTagsString=a|b|c  RConnTagsString=A|B|C  Frequency=50  Resistances="[ line(27,3)  line(27,3)*3]"  Inductances="[ line(27,4)  line(27,4)*3]"  Capacitances="[ line(27,5)  line(27,5)/3]"  Length=1
      settings: SourceProductName=Simscape Power Systems
  L-27-2 : powerlib/Elements/Three-Phase PI Section Line  LConnTagsString=a|b|c  RConnTagsString=A|B|C  Frequency=50  Resistances="[ line(27,3)  line(27,3)*3]"  Inductances="[ line(27,4)  line(27,4)*3]"  Capacitances="[ line(27,5)  line(27,5)/3]"  Length=1
      settings: SourceProductName=Simscape Power Systems
  L-28 : powerlib/Elements/Three-Phase PI Section Line  LConnTagsString=a|b|c  RConnTagsString=A|B|C  Frequency=50  Resistances="[ line(28,3)  line(28,3)*3]"  Inductances="[ line(28,4)  line(28,4)*3]"  Capacitances="[ line(28,5)  line(28,5)/3]"  Length=1
      settings: SourceProductName=Simscape Power Systems
  L-29-1 : powerlib/Elements/Three-Phase PI Section Line  LConnTagsString=a|b|c  RConnTagsString=A|B|C  Frequency=50  Resistances="[ line(29,3)  line(29,3)*3]"  Inductances="[ line(29,4)  line(29,4)*3]"  Capacitances="[ line(29,5)  line(29,5)/3]"  Length=1
      settings: SourceProductName=Simscape Power Systems
  L-29-2 : powerlib/Elements/Three-Phase PI Section Line  LConnTagsString=a|b|c  RConnTagsString=A|B|C  Frequency=50  Resistances="[ line(29,3)  line(29,3)*3]"  Inductances="[ line(29,4)  line(29,4)*3]"  Capacitances="[ line(29,5)  line(29,5)/3]"  Length=1
      settings: SourceProductName=Simscape Power Systems
  L-3-1 : powerlib/Elements/Three-Phase PI Section Line  LConnTagsString=a|b|c  RConnTagsString=A|B|C  Frequency=50  Resistances="[ line(3,3)  line(3,3)*3]"  Inductances="[ line(3,4)  line(3,4)*3]"  Capacitances="[ line(3,5)  line(3,5)/3]"  Length=1
      settings: SourceProductName=Simscape Power Systems
  L-3-2 : powerlib/Elements/Three-Phase PI Section Line  LConnTagsString=a|b|c  RConnTagsString=A|B|C  Frequency=50  Resistances="[ line(3,3)  line(3,3)*3]"  Inductances="[ line(3,4)  line(3,4)*3]"  Capacitances="[ line(3,5)  line(3,5)/3]"  Length=1
      settings: SourceProductName=Simscape Power Systems
  L-30-1 : powerlib/Elements/Three-Phase PI Section Line  LConnTagsString=a|b|c  RConnTagsString=A|B|C  Frequency=50  Resistances="[ line(30,3)  line(30,3)*3]"  Inductances="[ line(30,4)  line(30,4)*3]"  Capacitances="[ line(30,5)  line(30,5)/3]"  Length=1
      settings: SourceProductName=Simscape Power Systems
  L-30-2 : powerlib/Elements/Three-Phase PI Section Line  LConnTagsString=a|b|c  RConnTagsString=A|B|C  Frequency=50  Resistances="[ line(30,3)  line(30,3)*3]"  Inductances="[ line(30,4)  line(30,4)*3]"  Capacitances="[ line(30,5)  line(30,5)/3]"  Length=1
      settings: SourceProductName=Simscape Power Systems
  L-32 : powerlib/Elements/Three-Phase PI Section Line  LConnTagsString=a|b|c  RConnTagsString=A|B|C  Frequency=50  Resistances="[ line(32,3)  line(32,3)*3]"  Inductances="[ line(32,4)  line(32,4)*3]"  Capacitances="[ line(32,5)  line(32,5)/3]"  Length=1
      settings: SourceProductName=Simscape Power Systems
  L-33 : powerlib/Elements/Three-Phase PI Section Line  LConnTagsString=a|b|c  RConnTagsString=A|B|C  Frequency=50  Resistances="[ line(33,3)  line(33,3)*3]"  Inductances="[ line(33,4)  line(33,4)*3]"  Capacitances="[ line(33,5)  line(33,5)/3]"  Length=1
      settings: SourceProductName=Simscape Power Systems
  L-34-1 : powerlib/Elements/Three-Phase PI Section Line  LConnTagsString=a|b|c  RConnTagsString=A|B|C  Frequency=50  Resistances="[ line(34,3)  line(34,3)*3]"  Inductances="[ line(34,4)  line(34,4)*3]"  Capacitances="[ line(34,5)  line(34,5)/3]"  Length=1
      settings: SourceProductName=Simscape Power Systems
  L-34-2 : powerlib/Elements/Three-Phase PI Section Line  LConnTagsString=a|b|c  RConnTagsString=A|B|C  Frequency=50  Resistances="[ line(34,3)  line(34,3)*3]"  Inductances="[ line(34,4)  line(34,4)*3]"  Capacitances="[ line(34,5)  line(34,5)/3]"  Length=1
      settings: SourceProductName=Simscape Power Systems
  L-35-1 : powerlib/Elements/Three-Phase PI Section Line  LConnTagsString=a|b|c  RConnTagsString=A|B|C  Frequency=50  Resistances="[ line(35,3)  line(35,3)*3]"  Inductances="[ line(35,4)  line(35,4)*3]"  Capacitances="[ line(35,5)  line(35,5)/3]"  Length=1
      settings: SourceProductName=Simscape Power Systems
  L-35-2 : powerlib/Elements/Three-Phase PI Section Line  LConnTagsString=a|b|c  RConnTagsString=A|B|C  Frequency=50  Resistances="[ line(35,3)  line(35,3)*3]"  Inductances="[ line(35,4)  line(35,4)*3]"  Capacitances="[ line(35,5)  line(35,5)/3]"  Length=1
      settings: SourceProductName=Simscape Power Systems
  L-36-1 : powerlib/Elements/Three-Phase PI Section Line  LConnTagsString=a|b|c  RConnTagsString=A|B|C  Frequency=50  Resistances="[ line(36,3)  line(36,3)*3]"  Inductances="[ line(36,4)  line(36,4)*3]"  Capacitances="[ line(36,5)  line(36,5)/3]"  Length=1
      settings: SourceProductName=Simscape Power Systems
  L-37-1 : powerlib/Elements/Three-Phase PI Section Line  LConnTagsString=a|b|c  RConnTagsString=A|B|C  Frequency=50  Resistances="[ line(37,3)  line(37,3)*3]"  Inductances="[ line(37,4)  line(37,4)*3]"  Capacitances="[ line(37,5)  line(37,5)/3]"  Length=1
      settings: SourceProductName=Simscape Power Systems
  L-37-2 : powerlib/Elements/Three-Phase PI Section Line  LConnTagsString=a|b|c  RConnTagsString=A|B|C  Frequency=50  Resistances="[ line(37,3)  line(37,3)*3]"  Inductances="[ line(37,4)  line(37,4)*3]"  Capacitances="[ line(37,5)  line(37,5)/3]"  Length=1
      settings: SourceProductName=Simscape Power Systems
  L-37-3 : powerlib/Elements/Three-Phase PI Section Line  LConnTagsString=a|b|c  RConnTagsString=A|B|C  Frequency=50  Resistances="[ line(37,3)  line(37,3)*3]"  Inductances="[ line(37,4)  line(37,4)*3]"  Capacitances="[ line(37,5)  line(37,5)/3]"  Length=1
      settings: SourceProductName=Simscape Power Systems
  L-38-1 : powerlib/Elements/Three-Phase PI Section Line  LConnTagsString=a|b|c  RConnTagsString=A|B|C  Frequency=50  Resistances="[ line(38,3)  line(38,3)*3]"  Inductances="[ line(38,4)  line(38,4)*3]"  Capacitances="[ line(38,5)  line(38,5)/3]"  Length=1
      settings: SourceProductName=Simscape Power Systems
  L-38-2 : powerlib/Elements/Three-Phase PI Section Line  LConnTagsString=a|b|c  RConnTagsString=A|B|C  Frequency=50  Resistances="[ line(38,3)  line(38,3)*3]"  Inductances="[ line(38,4)  line(38,4)*3]"  Capacitances="[ line(38,5)  line(38,5)/3]"  Length=1
      settings: SourceProductName=Simscape Power Systems
  L-39 : powerlib/Elements/Three-Phase PI Section Line  LConnTagsString=a|b|c  RConnTagsString=A|B|C  Frequency=50  Resistances="[ line(39,3)  line(39,3)*3]"  Inductances="[ line(39,4)  line(39,4)*3]"  Capacitances="[ line(39,5)  line(39,5)/3]"  Length=1
      settings: SourceProductName=Simscape Power Systems
  L-4 : powerlib/Elements/Three-Phase PI Section Line  LConnTagsString=a|b|c  RConnTagsString=A|B|C  Frequency=50  Resistances="[ line(4,3)  line(4,3)*3]"  Inductances="[ line(4,4)  line(4,4)*3]"  Capacitances="[ line(4,5)  line(4,5)/3]"  Length=1
      settings: SourceProductName=Simscape Power Systems
  L-40-1 : powerlib/Elements/Three-Phase PI Section Line  LConnTagsString=a|b|c  RConnTagsString=A|B|C  Frequency=50  Resistances="[ line(40,3)  line(40,3)*3]"  Inductances="[ line(40,4)  line(40,4)*3]"  Capacitances="[ line(40,5)  line(40,5)/3]"  Length=1
      settings: SourceProductName=Simscape Power Systems
  L-40-2 : powerlib/Elements/Three-Phase PI Section Line  LConnTagsString=a|b|c  RConnTagsString=A|B|C  Frequency=50  Resistances="[ line(40,3)  line(40,3)*3]"  Inductances="[ line(40,4)  line(40,4)*3]"  Capacitances="[ line(40,5)  line(40,5)/3]"  Length=1
      settings: SourceProductName=Simscape Power Systems
  L-41-1 : powerlib/Elements/Three-Phase PI Section Line  LConnTagsString=a|b|c  RConnTagsString=A|B|C  Frequency=50  Resistances="[ line(41,3)  line(41,3)*3]"  Inductances="[ line(41,4)  line(41,4)*3]"  Capacitances="[ line(41,5)  line(41,5)/3]"  Length=1
      settings: SourceProductName=Simscape Power Systems
  L-41-2 : powerlib/Elements/Three-Phase PI Section Line  LConnTagsString=a|b|c  RConnTagsString=A|B|C  Frequency=50  Resistances="[ line(41,3)  line(41,3)*3]"  Inductances="[ line(41,4)  line(41,4)*3]"  Capacitances="[ line(41,5)  line(41,5)/3]"  Length=1
      settings: SourceProductName=Simscape Power Systems
  L-42 : powerlib/Elements/Three-Phase PI Section Line  LConnTagsString=a|b|c  RConnTagsString=A|B|C  Frequency=50  Resistances="[ line(42,3)  line(42,3)*3]"  Inductances="[ line(42,4)  line(42,4)*3]"  Capacitances="[ line(42,5)  line(42,5)/3]"  Length=1
      settings: SourceProductName=Simscape Power Systems
  L-43-{1..4} (4 alike) : powerlib/Elements/Three-Phase PI Section Line  LConnTagsString=a|b|c  RConnTagsString=A|B|C  Frequency=50  Resistances="[ line(43,3)  line(43,3)*3]"  Inductances="[ line(43,4)  line(43,4)*3]"  Capacitances="[ line(43,5)  line(43,5)/3]"  Length=1
      settings: SourceProductName=Simscape Power Systems
  L-44-1 : powerlib/Elements/Three-Phase PI Section Line  LConnTagsString=a|b|c  RConnTagsString=A|B|C  Frequency=50  Resistances="[ line(44,3)  line(44,3)*3]"  Inductances="[ line(44,4)  line(44,4)*3]"  Capacitances="[ line(44,5)  line(44,5)/3]"  Length=1
      settings: SourceProductName=Simscape Power Systems
  L-44-2 : powerlib/Elements/Three-Phase PI Section Line  LConnTagsString=a|b|c  RConnTagsString=A|B|C  Frequency=50  Resistances="[ line(44,3)  line(44,3)*3]"  Inductances="[ line(44,4)  line(44,4)*3]"  Capacitances="[ line(44,5)  line(44,5)/3]"  Length=1
      settings: SourceProductName=Simscape Power Systems
  L-45-1 : powerlib/Elements/Three-Phase PI Section Line  LConnTagsString=a|b|c  RConnTagsString=A|B|C  Frequency=50  Resistances="[ line(45,3)  line(45,3)*3]"  Inductances="[ line(45,4)  line(45,4)*3]"  Capacitances="[ line(45,5)  line(45,5)/3]"  Length=1
      settings: SourceProductName=Simscape Power Systems
  L-45-2 : powerlib/Elements/Three-Phase PI Section Line  LConnTagsString=a|b|c  RConnTagsString=A|B|C  Frequency=50  Resistances="[ line(45,3)  line(45,3)*3]"  Inductances="[ line(45,4)  line(45,4)*3]"  Capacitances="[ line(45,5)  line(45,5)/3]"  Length=1
      settings: SourceProductName=Simscape Power Systems
  L-46-1 : powerlib/Elements/Three-Phase PI Section Line  LConnTagsString=a|b|c  RConnTagsString=A|B|C  Frequency=50  Resistances="[ line(46,3)  line(46,3)*3]"  Inductances="[ line(46,4)  line(46,4)*3]"  Capacitances="[ line(46,5)  line(46,5)/3]"  Length=1
      settings: SourceProductName=Simscape Power Systems
  L-46-2 : powerlib/Elements/Three-Phase PI Section Line  LConnTagsString=a|b|c  RConnTagsString=A|B|C  Frequency=50  Resistances="[ line(46,3)  line(46,3)*3]"  Inductances="[ line(46,4)  line(46,4)*3]"  Capacitances="[ line(46,5)  line(46,5)/3]"  Length=1
      settings: SourceProductName=Simscape Power Systems
  L-47-1 : powerlib/Elements/Three-Phase PI Section Line  LConnTagsString=a|b|c  RConnTagsString=A|B|C  Frequency=50  Resistances="[ line(47,3)  line(47,3)*3]"  Inductances="[ line(47,4)  line(47,4)*3]"  Capacitances="[ line(47,5)  line(47,5)/3]"  Length=1
      settings: SourceProductName=Simscape Power Systems
  L-47-2 : powerlib/Elements/Three-Phase PI Section Line  LConnTagsString=a|b|c  RConnTagsString=A|B|C  Frequency=50  Resistances="[ line(47,3)  line(47,3)*3]"  Inductances="[ line(47,4)  line(47,4)*3]"  Capacitances="[ line(47,5)  line(47,5)/3]"  Length=1
      settings: SourceProductName=Simscape Power Systems
  L-48-1 : powerlib/Elements/Three-Phase PI Section Line  LConnTagsString=a|b|c  RConnTagsString=A|B|C  Frequency=50  Resistances="[ line(48,3)  line(48,3)*3]"  Inductances="[ line(48,4)  line(48,4)*3]"  Capacitances="[ line(48,5)  line(48,5)/3]"  Length=1
      settings: SourceProductName=Simscape Power Systems
  L-48-2 : powerlib/Elements/Three-Phase PI Section Line  LConnTagsString=a|b|c  RConnTagsString=A|B|C  Frequency=50  Resistances="[ line(48,3)  line(48,3)*3]"  Inductances="[ line(48,4)  line(48,4)*3]"  Capacitances="[ line(48,5)  line(48,5)/3]"  Length=1
      settings: SourceProductName=Simscape Power Systems
  L-49-1 : powerlib/Elements/Three-Phase PI Section Line  LConnTagsString=a|b|c  RConnTagsString=A|B|C  Frequency=50  Resistances="[ line(49,3)  line(49,3)*3]"  Inductances="[ line(49,4)  line(49,4)*3]"  Capacitances="[ line(49,5)  line(49,5)/3]"  Length=1
      settings: SourceProductName=Simscape Power Systems
  L-49-2 : powerlib/Elements/Three-Phase PI Section Line  LConnTagsString=a|b|c  RConnTagsString=A|B|C  Frequency=50  Resistances="[ line(49,3)  line(49,3)*3]"  Inductances="[ line(49,4)  line(49,4)*3]"  Capacitances="[ line(49,5)  line(49,5)/3]"  Length=1
      settings: SourceProductName=Simscape Power Systems
  L-5-1 : powerlib/Elements/Three-Phase PI Section Line  LConnTagsString=a|b|c  RConnTagsString=A|B|C  Frequency=50  Resistances="[ line(5,3)  line(5,3)*3]"  Inductances="[ line(5,4)  line(5,4)*3]"  Capacitances="[ line(5,5)  line(5,5)/3]"  Length=1
      settings: SourceProductName=Simscape Power Systems
  L-5-2 : powerlib/Elements/Three-Phase PI Section Line  LConnTagsString=a|b|c  RConnTagsString=A|B|C  Frequency=50  Resistances="[ line(5,3)  line(5,3)*3]"  Inductances="[ line(5,4)  line(5,4)*3]"  Capacitances="[ line(5,5)  line(5,5)/3]"  Length=1
      settings: SourceProductName=Simscape Power Systems
  L-50-1 : powerlib/Elements/Three-Phase PI Section Line  LConnTagsString=a|b|c  RConnTagsString=A|B|C  Frequency=50  Resistances="[ line(50,3)  line(50,3)*3]"  Inductances="[ line(50,4)  line(50,4)*3]"  Capacitances="[ line(50,5)  line(50,5)/3]"  Length=1
      settings: SourceProductName=Simscape Power Systems
  L-51 : powerlib/Elements/Three-Phase PI Section Line  LConnTagsString=a|b|c  RConnTagsString=A|B|C  Frequency=50  Resistances="[ line(51,3)  line(51,3)*3]"  Inductances="[ line(51,4)  line(51,4)*3]"  Capacitances="[ line(51,5)  line(51,5)/3]"  Length=1
      settings: SourceProductName=Simscape Power Systems
  L-52 : powerlib/Elements/Three-Phase PI Section Line  LConnTagsString=a|b|c  RConnTagsString=A|B|C  Frequency=50  Resistances="[ line(52,3)  line(52,3)*3]"  Inductances="[ line(52,4)  line(52,4)*3]"  Capacitances="[ line(52,5)  line(52,5)/3]"  Length=1
      settings: SourceProductName=Simscape Power Systems
  L-53 : powerlib/Elements/Three-Phase PI Section Line  LConnTagsString=a|b|c  RConnTagsString=A|B|C  Frequency=50  Resistances="[ line(53,3)  line(53,3)*3]"  Inductances="[ line(53,4)  line(53,4)*3]"  Capacitances="[ line(53,5)  line(53,5)/3]"  Length=1
      settings: SourceProductName=Simscape Power Systems
  L-54 : powerlib/Elements/Three-Phase PI Section Line  LConnTagsString=a|b|c  RConnTagsString=A|B|C  Frequency=50  Resistances=[ line(54,3) line(54,3)*3]  Inductances=[ line(54,4) line(54,4)*3]  Capacitances=[ line(54,5) line(54,5)/3]  Length=1
      settings: SourceProductName=Simscape Power Systems
  L-55-1 : powerlib/Elements/Three-Phase PI Section Line  LConnTagsString=a|b|c  RConnTagsString=A|B|C  Frequency=50  Resistances=[ line(55,3) line(55,3)*3]  Inductances="[ line(55,4)  line(55,4)*3]"  Capacitances="[line(55,5)  line(55,5)/3]"  Length=1
      settings: SourceProductName=Simscape Power Systems
  L-55-2 : powerlib/Elements/Three-Phase PI Section Line  LConnTagsString=a|b|c  RConnTagsString=A|B|C  Frequency=50  Resistances=[ line(55,3) line(55,3)*3]  Inductances="[ line(55,4)  line(55,4)*3]"  Capacitances="[line(55,5)  line(55,5)/3]"  Length=1
      settings: SourceProductName=Simscape Power Systems
  L-6-1 : powerlib/Elements/Three-Phase PI Section Line  LConnTagsString=a|b|c  RConnTagsString=A|B|C  Frequency=50  Resistances="[ line(6,3)  line(6,3)*3]"  Inductances="[ line(6,4)  line(6,4)*3]"  Capacitances="[ line(6,5)  line(6,5)/3]"  Length=1
      settings: SourceProductName=Simscape Power Systems
  L-6-2 : powerlib/Elements/Three-Phase PI Section Line  LConnTagsString=a|b|c  RConnTagsString=A|B|C  Frequency=50  Resistances="[ line(6,3)  line(6,3)*3]"  Inductances="[ line(6,4)  line(6,4)*3]"  Capacitances="[ line(6,5)  line(6,5)/3]"  Length=1
      settings: SourceProductName=Simscape Power Systems
  L-7-1 : powerlib/Elements/Three-Phase PI Section Line  LConnTagsString=a|b|c  RConnTagsString=A|B|C  Frequency=50  Resistances="[ line(7,3)  line(7,3)*3]"  Inductances="[ line(7,4)  line(7,4)*3]"  Capacitances="[ line(7,5)  line(7,5)/3]"  Length=1
      settings: SourceProductName=Simscape Power Systems
  L-7-2 : powerlib/Elements/Three-Phase PI Section Line  LConnTagsString=a|b|c  RConnTagsString=A|B|C  Frequency=50  Resistances="[ line(7,3)  line(7,3)*3]"  Inductances="[ line(7,4)  line(7,4)*3]"  Capacitances="[ line(7,5)  line(7,5)/3]"  Length=1
      settings: SourceProductName=Simscape Power Systems
  L-8-1 : powerlib/Elements/Three-Phase PI Section Line  LConnTagsString=a|b|c  RConnTagsString=A|B|C  Frequency=50  Resistances="[ line(8,3)  line(8,3)*3]"  Inductances="[ line(8,4)  line(8,4)*3]"  Capacitances="[ line(8,5)  line(8,5)/3]"  Length=1
      settings: SourceProductName=Simscape Power Systems
  L-8-2 : powerlib/Elements/Three-Phase PI Section Line  LConnTagsString=a|b|c  RConnTagsString=A|B|C  Frequency=50  Resistances="[ line(8,3)  line(8,3)*3]"  Inductances="[ line(8,4)  line(8,4)*3]"  Capacitances="[ line(8,5)  line(8,5)/3]"  Length=1
      settings: SourceProductName=Simscape Power Systems
  L-9-1 : powerlib/Elements/Three-Phase PI Section Line  LConnTagsString=a|b|c  RConnTagsString=A|B|C  Frequency=50  Resistances="[ line(9,3)  line(9,3)*3]"  Inductances="[ line(9,4)  line(9,4)*3]"  Capacitances="[ line(9,5)  line(9,5)/3]"  Length=1
      settings: SourceProductName=Simscape Power Systems
  L-9-2 : powerlib/Elements/Three-Phase PI Section Line  LConnTagsString=a|b|c  RConnTagsString=A|B|C  Frequency=50  Resistances="[ line(9,3)  line(9,3)*3]"  Inductances="[ line(9,4)  line(9,4)*3]"  Capacitances="[ line(9,5)  line(9,5)/3]"  Length=1
      settings: SourceProductName=Simscape Power Systems
  Load Flow Bus10 : powerlib/Measurements/Load Flow Bus  LConnTagsString=a  Phases=single  Connectors=on one side  ID=B301  Vbase=20e3  Vref=1  Vangle=0  VLF=1  VLFb=1  VLFc=1  angleLF=-10.04  angleLFb=0  angleLFc=0
      settings: AttributesFormatString=%<ID>\n%<Vbase>V\n%<VLF>pu\n%<angleLF>deg.  SourceProductName=Simscape Power Systems
  Load Flow Bus11 : powerlib/Measurements/Load Flow Bus  LConnTagsString=a  Phases=single  Connectors=on one side  ID=B302  Vbase=20e3  Vref=1  Vangle=0  VLF=1  VLFb=1  VLFc=1  angleLF=-18.96  angleLFb=0  angleLFc=0
      settings: AttributesFormatString=%<ID>\n%<Vbase>V\n%<VLF>pu\n%<angleLF>deg.  SourceProductName=Simscape Power Systems
  Load Flow Bus12 : powerlib/Measurements/Load Flow Bus  LConnTagsString=a  Phases=single  Connectors=on one side  ID=B503  Vbase=15e3  Vref=1  Vangle=0  VLF=1  VLFb=1  VLFc=1  angleLF=-38.47  angleLFb=0  angleLFc=0
      settings: AttributesFormatString=%<ID>\n%<Vbase>V\n%<VLF>pu\n%<angleLF>deg.  SourceProductName=Simscape Power Systems
  Load Flow Bus13 : powerlib/Measurements/Load Flow Bus  LConnTagsString=a  Phases=single  Connectors=on one side  ID=B502  Vbase=15e3  Vref=1  Vangle=0  VLF=0.9992  VLFb=1  VLFc=1  angleLF=-2.878  angleLFb=0  angleLFc=0
      settings: AttributesFormatString=%<ID>\n%<Vbase>V\n%<VLF>pu\n%<angleLF>deg.  SourceProductName=Simscape Power Systems
  Load Flow Bus14 : powerlib/Measurements/Load Flow Bus  LConnTagsString=a  Phases=single  Connectors=on one side  ID=B501  Vbase=20e3  Vref=1  Vangle=0  VLF=1  VLFb=1  VLFc=1  angleLF=-34.56  angleLFb=0  angleLFc=0
      settings: AttributesFormatString=%<ID>\n%<Vbase>V\n%<VLF>pu\n%<angleLF>deg.  SourceProductName=Simscape Power Systems
  Load Flow Bus15 : powerlib/Measurements/Load Flow Bus  LConnTagsString=a  Phases=single  Connectors=on one side  ID=B403  Vbase=20e3  Vref=1  Vangle=0  VLF=0.9972  VLFb=1  VLFc=1  angleLF=23.58  angleLFb=0  angleLFc=0
      settings: AttributesFormatString=%<ID>\n%<Vbase>V\n%<VLF>pu\n%<angleLF>deg.  SourceProductName=Simscape Power Systems
  Load Flow Bus2 : powerlib/Measurements/Load Flow Bus  LConnTagsString=a  Phases=single  Connectors=on one side  ID=B404  Vbase=20e3  Vref=1  Vangle=0  VLF=1  VLFb=1  VLFc=1  angleLF=-13.1  angleLFb=0  angleLFc=0
      settings: AttributesFormatString=%<ID>\n%<Vbase>V\n%<VLF>pu\n%<angleLF>deg.  SourceProductName=Simscape Power Systems
  Load Flow Bus3 : powerlib/Measurements/Load Flow Bus  LConnTagsString=a  Phases=single  Connectors=on one side  ID=B402  Vbase=20e3  Vref=1  Vangle=0  VLF=0.9966  VLFb=1  VLFc=1  angleLF=23.92  angleLFb=0  angleLFc=0
      settings: AttributesFormatString=%<ID>\n%<Vbase>V\n%<VLF>pu\n%<angleLF>deg.  SourceProductName=Simscape Power Systems
  Load Flow Bus4 : powerlib/Measurements/Load Flow Bus  LConnTagsString=a  Phases=single  Connectors=on one side  ID=B401  Vbase=20e3  Vref=1  Vangle=0  VLF=1  VLFb=1  VLFc=1  angleLF=-21.06  angleLFb=0  angleLFc=0
      settings: AttributesFormatString=%<ID>\n%<Vbase>V\n%<VLF>pu\n%<angleLF>deg.  SourceProductName=Simscape Power Systems
  Load Flow Bus5 : powerlib/Measurements/Load Flow Bus  LConnTagsString=a  Phases=single  Connectors=on one side  ID=B203  Vbase=20e3  Vref=1  Vangle=0  VLF=1  VLFb=1  VLFc=1  angleLF=-0.543  angleLFb=0  angleLFc=0
      settings: AttributesFormatString=%<ID>\n%<Vbase>V\n%<VLF>pu\n%<angleLF>deg.  SourceProductName=Simscape Power Systems
  Load Flow Bus6 : powerlib/Measurements/Load Flow Bus  LConnTagsString=a  Phases=single  Connectors=on one side  ID=B201  Vbase=20e3  Vref=1  Vangle=0  VLF=1  VLFb=1  VLFc=1  angleLF=3.923  angleLFb=0  angleLFc=0
      settings: AttributesFormatString=%<ID>\n%<Vbase>V\n%<VLF>pu\n%<angleLF>deg.  SourceProductName=Simscape Power Systems
  Load Flow Bus7 : powerlib/Measurements/Load Flow Bus  LConnTagsString=a  Phases=single  Connectors=on one side  ID=B202  Vbase=20e3  Vref=1  Vangle=0  VLF=1  VLFb=1  VLFc=1  angleLF=-0.2053  angleLFb=0  angleLFc=0
      settings: AttributesFormatString=%<ID>\n%<Vbase>V\n%<VLF>pu\n%<angleLF>deg.  SourceProductName=Simscape Power Systems
  Load Flow Bus8 : powerlib/Measurements/Load Flow Bus  LConnTagsString=a  Phases=single  Connectors=on one side  ID=B204  Vbase=20e3  Vref=1  Vangle=0  VLF=1  VLFb=1  VLFc=1  angleLF=0  angleLFb=0  angleLFc=0
      settings: AttributesFormatString=%<ID>\n%<Vbase>V\n%<VLF>pu\n%<angleLF>deg.  SourceProductName=Simscape Power Systems
  Load Flow Bus9 : powerlib/Measurements/Load Flow Bus  LConnTagsString=a  Phases=single  Connectors=on one side  ID=B101  Vbase=15e3  Vref=1  Vangle=0  VLF=1.083  VLFb=1  VLFc=1  angleLF=6.603  angleLFb=0  angleLFc=0
      settings: AttributesFormatString=%<ID>\n%<Vbase>V\n%<VLF>pu\n%<angleLF>deg.  SourceProductName=Simscape Power Systems
  Load1 : powerlib/Elements/Three-Phase Parallel RLC Load  LConnTagsString=A|B|C  Configuration=Y (grounded)  NominalVoltage=(356540)*1.00295  Vabc=[1e3 1e3 1e3]  Vabcp=[1e3 1e3 1e3]  NominalFrequency=50  UnbalancedPower=off  ActivePower=load_mag(1,2)*1e6  InductivePower=load_mag(1,3)*1e6  CapacitivePower=0  Pabc=[10e3 9e3 11e3]  QLabc=[100 90 110]  QCabc=[100 90 110]  Pabcp=[10e3 9e3 11e3]  QLabcp=[100 90 110]  QCabcp=[100 90 110]  Measurements=None  LoadType=constant PQ
  Load10 : powerlib/Elements/Three-Phase Parallel RLC Load  LConnTagsString=A|B|C  Configuration=Y (grounded)  NominalVoltage=(346286)*1.00201  Vabc=[1e3 1e3 1e3]  Vabcp=[1e3 1e3 1e3]  NominalFrequency=50  UnbalancedPower=off  ActivePower=load_mag(10,2)*1e6  InductivePower=load_mag(10,3)*1e6  CapacitivePower=0  Pabc=[10e3 9e3 11e3]  QLabc=[100 90 110]  QCabc=[100 90 110]  Pabcp=[10e3 9e3 11e3]  QLabcp=[100 90 110]  QCabcp=[100 90 110]  Measurements=None  LoadType=constant PQ
  Load11 : powerlib/Elements/Three-Phase Parallel RLC Load  LConnTagsString=A|B|C  Configuration=Y (grounded)  NominalVoltage=(511149)*1.0019  Vabc=[1e3 1e3 1e3]  Vabcp=[1e3 1e3 1e3]  NominalFrequency=50  UnbalancedPower=off  ActivePower=load_mag(11,2)*1e6  InductivePower=load_mag(11,3)*1e6  CapacitivePower=0  Pabc=[10e3 9e3 11e3]  QLabc=[100 90 110]  QCabc=[100 90 110]  Pabcp=[10e3 9e3 11e3]  QLabcp=[100 90 110]  QCabcp=[100 90 110]  Measurements=None  LoadType=constant PQ
  Load12 : powerlib/Elements/Three-Phase Parallel RLC Load  LConnTagsString=A|B|C  Configuration=Y (grounded)  NominalVoltage=(512503)*1.00192  Vabc=[1e3 1e3 1e3]  Vabcp=[1e3 1e3 1e3]  NominalFrequency=50  UnbalancedPower=off  ActivePower=load_mag(12,2)*1e6  InductivePower=load_mag(12,3)*1e6  CapacitivePower=0  Pabc=[10e3 9e3 11e3]  QLabc=[100 90 110]  QCabc=[100 90 110]  Pabcp=[10e3 9e3 11e3]  QLabcp=[100 90 110]  QCabcp=[100 90 110]  Measurements=None  LoadType=constant PQ
  Load13 : powerlib/Elements/Three-Phase Parallel RLC Load  LConnTagsString=A|B|C  Configuration=Y (grounded)  NominalVoltage=(529566)*1.00301  Vabc=[1e3 1e3 1e3]  Vabcp=[1e3 1e3 1e3]  NominalFrequency=50  UnbalancedPower=off  ActivePower=load_mag(13,2)*1e6  InductivePower=load_mag(13,3)*1e6  CapacitivePower=0  Pabc=[10e3 9e3 11e3]  QLabc=[100 90 110]  QCabc=[100 90 110]  Pabcp=[10e3 9e3 11e3]  QLabcp=[100 90 110]  QCabcp=[100 90 110]  Measurements=None  LoadType=constant PQ
  Load14 : powerlib/Elements/Three-Phase Parallel RLC Load  LConnTagsString=A|B|C  Configuration=Y (grounded)  NominalVoltage=(357825)*1.00308  Vabc=[1e3 1e3 1e3]  Vabcp=[1e3 1e3 1e3]  NominalFrequency=50  UnbalancedPower=off  ActivePower=load_mag(14,2)*1e6  InductivePower=load_mag(14,3)*1e6  CapacitivePower=0  Pabc=[10e3 9e3 11e3]  QLabc=[100 90 110]  QCabc=[100 90 110]  Pabcp=[10e3 9e3 11e3]  QLabcp=[100 90 110]  QCabcp=[100 90 110]  Measurements=None  LoadType=constant PQ
  Load15 : powerlib/Elements/Three-Phase Parallel RLC Load  LConnTagsString=A|B|C  Configuration=Y (grounded)  NominalVoltage=(220026)*1.00158  Vabc=[1e3 1e3 1e3]  Vabcp=[1e3 1e3 1e3]  NominalFrequency=50  UnbalancedPower=off  ActivePower=load_mag(15,2)*1e6  InductivePower=load_mag(15,3)*1e6  CapacitivePower=0  Pabc=[10e3 9e3 11e3]  QLabc=[100 90 110]  QCabc=[100 90 110]  Pabcp=[10e3 9e3 11e3]  QLabcp=[100 90 110]  QCabcp=[100 90 110]  Measurements=None  LoadType=constant PQ
  Load16 : powerlib/Elements/Three-Phase Parallel RLC Load  LConnTagsString=A|B|C  Configuration=Y (grounded)  NominalVoltage=(218962)*1.00201  Vabc=[1e3 1e3 1e3]  Vabcp=[1e3 1e3 1e3]  NominalFrequency=50  UnbalancedPower=off  ActivePower=load_mag(16,2)*1e6  InductivePower=load_mag(16,3)*1e6  CapacitivePower=0  Pabc=[10e3 9e3 11e3]  QLabc=[100 90 110]  QCabc=[100 90 110]  Pabcp=[10e3 9e3 11e3]  QLabcp=[100 90 110]  QCabcp=[100 90 110]  Measurements=None  LoadType=constant PQ
  Load17 : powerlib/Elements/Three-Phase Parallel RLC Load  LConnTagsString=A|B|C  Configuration=Y (grounded)  NominalVoltage=(220626)*1.00218  Vabc=[1e3 1e3 1e3]  Vabcp=[1e3 1e3 1e3]  NominalFrequency=50  UnbalancedPower=off  ActivePower=load_mag(17,2)*1e6  InductivePower=load_mag(17,3)*1e6  CapacitivePower=0  Pabc=[10e3 9e3 11e3]  QLabc=[100 90 110]  QCabc=[100 90 110]  Pabcp=[10e3 9e3 11e3]  QLabcp=[100 90 110]  QCabcp=[100 90 110]  Measurements=None  LoadType=constant PQ
  Load18 : powerlib/Elements/Three-Phase Parallel RLC Load  LConnTagsString=A|B|C  Configuration=Y (grounded)  NominalVoltage=(276748)*1.00132  Vabc=[1e3 1e3 1e3]  Vabcp=[1e3 1e3 1e3]  NominalFrequency=50  UnbalancedPower=off  ActivePower=load_mag(18,2)*1e6  InductivePower=load_mag(18,3)*1e6  CapacitivePower=0  Pabc=[10e3 9e3 11e3]  QLabc=[100 90 110]  QCabc=[100 90 110]  Pabcp=[10e3 9e3 11e3]  QLabcp=[100 90 110]  QCabcp=[100 90 110]  Measurements=None  LoadType=constant PQ
  Load19 : powerlib/Elements/Three-Phase Parallel RLC Load  LConnTagsString=A|B|C  Configuration=Y (grounded)  NominalVoltage=(273917)*1.00148  Vabc=[1e3 1e3 1e3]  Vabcp=[1e3 1e3 1e3]  NominalFrequency=50  UnbalancedPower=off  ActivePower=load_mag(19,2)*1e6  InductivePower=load_mag(19,3)*1e6  CapacitivePower=0  Pabc=[10e3 9e3 11e3]  QLabc=[100 90 110]  QCabc=[100 90 110]  Pabcp=[10e3 9e3 11e3]  QLabcp=[100 90 110]  QCabcp=[100 90 110]  Measurements=None  LoadType=constant PQ
  Load2 : powerlib/Elements/Three-Phase Parallel RLC Load  LConnTagsString=A|B|C  Configuration=Y (grounded)  NominalVoltage=(346402)*1.00069  Vabc=[1e3 1e3 1e3]  Vabcp=[1e3 1e3 1e3]  NominalFrequency=50  UnbalancedPower=off  ActivePower=load_mag(2,2)*1e6  InductivePower=load_mag(2,3)*1e6  CapacitivePower=0  Pabc=[10e3 9e3 11e3]  QLabc=[100 90 110]  QCabc=[100 90 110]  Pabcp=[10e3 9e3 11e3]  QLabcp=[100 90 110]  QCabcp=[100 90 110]  Measurements=None  LoadType=constant PQ
  Load20 : powerlib/Elements/Three-Phase Parallel RLC Load  LConnTagsString=A|B|C  Configuration=Y (grounded)  NominalVoltage=(274336)*1.00148  Vabc=[1e3 1e3 1e3]  Vabcp=[1e3 1e3 1e3]  NominalFrequency=50  UnbalancedPower=off  ActivePower=load_mag(20,2)*1e6  InductivePower=load_mag(20,3)*1e6  CapacitivePower=0  Pabc=[10e3 9e3 11e3]  QLabc=[100 90 110]  QCabc=[100 90 110]  Pabcp=[10e3 9e3 11e3]  QLabcp=[100 90 110]  QCabcp=[100 90 110]  Measurements=None  LoadType=constant PQ
  Load21 : powerlib/Elements/Three-Phase Parallel RLC Load  LConnTagsString=A|B|C  Configuration=Y (grounded)  NominalVoltage=(277487)*1.0014  Vabc=[1e3 1e3 1e3]  Vabcp=[1e3 1e3 1e3]  NominalFrequency=50  UnbalancedPower=off  ActivePower=load_mag(21,2)*1e6  InductivePower=load_mag(21,3)*1e6  CapacitivePower=0  Pabc=[10e3 9e3 11e3]  QLabc=[100 90 110]  QCabc=[100 90 110]  Pabcp=[10e3 9e3 11e3]  QLabcp=[100 90 110]  QCabcp=[100 90 110]  Measurements=None  LoadType=constant PQ
  Load22 : powerlib/Elements/Three-Phase Parallel RLC Load  LConnTagsString=A|B|C  Configuration=Y (grounded)  NominalVoltage=(275000)*1.03603  Vabc=[1e3 1e3 1e3]  Vabcp=[1e3 1e3 1e3]  NominalFrequency=50  UnbalancedPower=off  ActivePower=load_mag(22,2)*1e6  InductivePower=load_mag(22,3)*1e6  CapacitivePower=0  Pabc=[10e3 9e3 11e3]  QLabc=[100 90 110]  QCabc=[100 90 110]  Pabcp=[10e3 9e3 11e3]  QLabcp=[100 90 110]  QCabcp=[100 90 110]  Measurements=None  LoadType=constant PQ
  Load23 : powerlib/Elements/Three-Phase Parallel RLC Load  LConnTagsString=A|B|C  Configuration=Y (grounded)  NominalVoltage=(278478)*1.00098  Vabc=[1e3 1e3 1e3]  Vabcp=[1e3 1e3 1e3]  NominalFrequency=50  UnbalancedPower=off  ActivePower=load_mag(23,2)*1e6  InductivePower=load_mag(23,3)*1e6  CapacitivePower=0  Pabc=[10e3 9e3 11e3]  QLabc=[100 90 110]  QCabc=[100 90 110]  Pabcp=[10e3 9e3 11e3]  QLabcp=[100 90 110]  QCabcp=[100 90 110]  Measurements=Branch voltages  LoadType=constant PQ
  Load24 : powerlib/Elements/Three-Phase Parallel RLC Load  LConnTagsString=A|B|C  Configuration=Y (grounded)  NominalVoltage=(275000)*1.01119  Vabc=[1e3 1e3 1e3]  Vabcp=[1e3 1e3 1e3]  NominalFrequency=50  UnbalancedPower=off  ActivePower=load_mag(24,2)*1e6  InductivePower=load_mag(24,3)*1e6  CapacitivePower=0  Pabc=[10e3 9e3 11e3]  QLabc=[100 90 110]  QCabc=[100 90 110]  Pabcp=[10e3 9e3 11e3]  QLabcp=[100 90 110]  QCabcp=[100 90 110]  Measurements=None  LoadType=constant PQ
  Load25 : powerlib/Elements/Three-Phase Parallel RLC Load  LConnTagsString=A|B|C  Configuration=Y (grounded)  NominalVoltage=(276329)*1.00111  Vabc=[1e3 1e3 1e3]  Vabcp=[1e3 1e3 1e3]  NominalFrequency=50  UnbalancedPower=off  ActivePower=load_mag(25,2)*1e6  InductivePower=load_mag(25,3)*1e6  CapacitivePower=0  Pabc=[10e3 9e3 11e3]  QLabc=[100 90 110]  QCabc=[100 90 110]  Pabcp=[10e3 9e3 11e3]  QLabcp=[100 90 110]  QCabcp=[100 90 110]  Measurements=None  LoadType=constant PQ
  Load26 : powerlib/Elements/Three-Phase Parallel RLC Load  LConnTagsString=A|B|C  Configuration=Y (grounded)  NominalVoltage=(285470)*1.00204  Vabc=[1e3 1e3 1e3]  Vabcp=[1e3 1e3 1e3]  NominalFrequency=50  UnbalancedPower=off  ActivePower=load_mag(26,2)*1e6  InductivePower=load_mag(26,3)*1e6  CapacitivePower=0  Pabc=[10e3 9e3 11e3]  QLabc=[100 90 110]  QCabc=[100 90 110]  Pabcp=[10e3 9e3 11e3]  QLabcp=[100 90 110]  QCabcp=[100 90 110]  Measurements=None  LoadType=constant PQ
  Load27 : powerlib/Elements/Three-Phase Parallel RLC Load  LConnTagsString=A|B|C  Configuration=Y (grounded)  NominalVoltage=(279067)*1.00215  Vabc=[1e3 1e3 1e3]  Vabcp=[1e3 1e3 1e3]  NominalFrequency=50  UnbalancedPower=off  ActivePower=load_mag(27,2)*1e6  InductivePower=load_mag(27,3)*1e6  CapacitivePower=0  Pabc=[10e3 9e3 11e3]  QLabc=[100 90 110]  QCabc=[100 90 110]  Pabcp=[10e3 9e3 11e3]  QLabcp=[100 90 110]  QCabcp=[100 90 110]  Measurements=None  LoadType=constant PQ
  Load28 : powerlib/Elements/Three-Phase Parallel RLC Load  LConnTagsString=A|B|C  Configuration=Y (grounded)  NominalVoltage=(277109)*1.00233  Vabc=[1e3 1e3 1e3]  Vabcp=[1e3 1e3 1e3]  NominalFrequency=50  UnbalancedPower=off  ActivePower=load_mag(28,2)*1e6  InductivePower=load_mag(28,3)*1e6  CapacitivePower=0  Pabc=[10e3 9e3 11e3]  QLabc=[100 90 110]  QCabc=[100 90 110]  Pabcp=[10e3 9e3 11e3]  QLabcp=[100 90 110]  QCabcp=[100 90 110]  Measurements=None  LoadType=constant PQ
  Load29 : powerlib/Elements/Three-Phase Parallel RLC Load  LConnTagsString=A|B|C  Configuration=Y (grounded)  NominalVoltage=(295429)*1.00282  Vabc=[1e3 1e3 1e3]  Vabcp=[1e3 1e3 1e3]  NominalFrequency=50  UnbalancedPower=off  ActivePower=load_mag(29,2)*1e6  InductivePower=load_mag(29,3)*1e6  CapacitivePower=0  Pabc=[10e3 9e3 11e3]  QLabc=[100 90 110]  QCabc=[100 90 110]  Pabcp=[10e3 9e3 11e3]  QLabcp=[100 90 110]  QCabcp=[100 90 110]  Measurements=None  LoadType=constant PQ
  Load3 : powerlib/Elements/Three-Phase Parallel RLC Load  LConnTagsString=A|B|C  Configuration=Y (grounded)  NominalVoltage=(335481)*1.00046  Vabc=[1e3 1e3 1e3]  Vabcp=[1e3 1e3 1e3]  NominalFrequency=50  UnbalancedPower=off  ActivePower=load_mag(3,2)*1e6  InductivePower=load_mag(3,3)*1e6  CapacitivePower=0  Pabc=[10e3 9e3 11e3]  QLabc=[100 90 110]  QCabc=[100 90 110]  Pabcp=[10e3 9e3 11e3]  QLabcp=[100 90 110]  QCabcp=[100 90 110]  Measurements=None  LoadType=constant PQ
  Load30 : powerlib/Elements/Three-Phase Parallel RLC Load  Commented=on  LConnTagsString=A|B|C  Configuration=Y (grounded)  NominalVoltage=trans(21,4)*1e3  Vabc=[1e3 1e3 1e3]  Vabcp=[1e3 1e3 1e3]  NominalFrequency=50  UnbalancedPower=off  ActivePower=p(14,3)*1e6*0.89982  InductivePower=0  CapacitivePower=0  Pabc=[10e3 9e3 11e3]  QLabc=[100 90 110]  QCabc=[100 90 110]  Pabcp=[10e3 9e3 11e3]  QLabcp=[100 90 110]  QCabcp=[100 90 110]  Measurements=None  LoadType=constant PQ
  Load4 : powerlib/Elements/Three-Phase Parallel RLC Load  LConnTagsString=A|B|C  Configuration=Y (grounded)  NominalVoltage=(331947)*1.00076  Vabc=[1e3 1e3 1e3]  Vabcp=[1e3 1e3 1e3]  NominalFrequency=50  UnbalancedPower=off  ActivePower=load_mag(4,2)*1e6  InductivePower=load_mag(4,3)*1e6  CapacitivePower=0  Pabc=[10e3 9e3 11e3]  QLabc=[100 90 110]  QCabc=[100 90 110]  Pabcp=[10e3 9e3 11e3]  QLabcp=[100 90 110]  QCabcp=[100 90 110]  Measurements=None  LoadType=constant PQ
  Load5 : powerlib/Elements/Three-Phase Parallel RLC Load  LConnTagsString=A|B|C  Configuration=Y (grounded)  NominalVoltage=(332888)*1.00092  Vabc=[1e3 1e3 1e3]  Vabcp=[1e3 1e3 1e3]  NominalFrequency=50  UnbalancedPower=off  ActivePower=load_mag(5,2)*1e6  InductivePower=load_mag(5,3)*1e6  CapacitivePower=0  Pabc=[10e3 9e3 11e3]  QLabc=[100 90 110]  QCabc=[100 90 110]  Pabcp=[10e3 9e3 11e3]  QLabcp=[100 90 110]  QCabcp=[100 90 110]  Measurements=None  LoadType=constant PQ
  Load6 : powerlib/Elements/Three-Phase Parallel RLC Load  LConnTagsString=A|B|C  Configuration=Y (grounded)  NominalVoltage=(335217)*1.0013  Vabc=[1e3 1e3 1e3]  Vabcp=[1e3 1e3 1e3]  NominalFrequency=50  UnbalancedPower=off  ActivePower=load_mag(6,2)*1e6  InductivePower=load_mag(6,3)*1e6  CapacitivePower=0  Pabc=[10e3 9e3 11e3]  QLabc=[100 90 110]  QCabc=[100 90 110]  Pabcp=[10e3 9e3 11e3]  QLabcp=[100 90 110]  QCabcp=[100 90 110]  Measurements=None  LoadType=constant PQ
  Load7 : powerlib/Elements/Three-Phase Parallel RLC Load  LConnTagsString=A|B|C  Configuration=Y (grounded)  NominalVoltage=(330000)*1.02708  Vabc=[1e3 1e3 1e3]  Vabcp=[1e3 1e3 1e3]  NominalFrequency=50  UnbalancedPower=off  ActivePower=load_mag(7,2)*1e6  InductivePower=load_mag(7,3)*1e6  CapacitivePower=0  Pabc=[10e3 9e3 11e3]  QLabc=[100 90 110]  QCabc=[100 90 110]  Pabcp=[10e3 9e3 11e3]  QLabcp=[100 90 110]  QCabcp=[100 90 110]  Measurements=None  LoadType=constant PQ
  Load8 : powerlib/Elements/Three-Phase Parallel RLC Load  LConnTagsString=A|B|C  Configuration=Y (grounded)  NominalVoltage=(335416)*1.00085  Vabc=[1e3 1e3 1e3]  Vabcp=[1e3 1e3 1e3]  NominalFrequency=50  UnbalancedPower=off  ActivePower=load_mag(8,2)*1e6  InductivePower=load_mag(8,3)*1e6  CapacitivePower=0  Pabc=[10e3 9e3 11e3]  QLabc=[100 90 110]  QCabc=[100 90 110]  Pabcp=[10e3 9e3 11e3]  QLabcp=[100 90 110]  QCabcp=[100 90 110]  Measurements=None  LoadType=constant PQ
  Load9 : powerlib/Elements/Three-Phase Parallel RLC Load  LConnTagsString=A|B|C  Configuration=Y (grounded)  NominalVoltage=(330000)*1.03661  Vabc=[1e3 1e3 1e3]  Vabcp=[1e3 1e3 1e3]  NominalFrequency=50  UnbalancedPower=off  ActivePower=load_mag(9,2)*1e6  InductivePower=load_mag(9,3)*1e6  CapacitivePower=0  Pabc=[10e3 9e3 11e3]  QLabc=[100 90 110]  QCabc=[100 90 110]  Pabcp=[10e3 9e3 11e3]  QLabcp=[100 90 110]  QCabcp=[100 90 110]  Measurements=None  LoadType=constant PQ
  Measurements_VI : Subsystem
  Measurements_low : Subsystem  Commented=on
  P 1-3 : Scope  NumInputPorts=2
  P 2-1 : Scope  NumInputPorts=2
  P 3-5 : Scope  NumInputPorts=2
  P 4-2 : Scope  NumInputPorts=2
  PSS model : Constant  Value=PSSMODEL
  Scope : Scope
  T1 : powerlib/Elements/Three-Phase Transformer (Two Windings)  Winding1Connection=Yg  Winding2Connection=Yg  CoreType=Three single-phase transformers  SetSaturation=off  Hysteresis=off  DataFile='hysteresis'  SetInitialFlux=off  Measurements=None  UNITS=pu  NominalPower=[ trans(1,6)*1e6 , 50 ]  Winding1=[ trans(1,4)*1e3, 1e-6, 0 ]  Winding2=[ trans(1,5)*1e3, 1e-6, trans(1,7) ]  Rm=500  Lm=500  L0=0.5  Saturation=[ 0,0 ; 0.0024,1.2 ; 1.0,1.52 ]  InitialFluxes=[ 0.8 , -0.8 , 0.7 ]  MoreParameters=off  BreakLoop=off  DataType=off  TransfoNumber=0
  T10 : powerlib/Elements/Three-Phase Transformer (Two Windings)  Winding1Connection=Y  Winding2Connection=Y  CoreType=Three single-phase transformers  SetSaturation=off  Hysteresis=off  DataFile='hysteresis'  SetInitialFlux=off  Measurements=None  UNITS=pu  NominalPower=[ trans(10,6)*1e6 , 50 ]  Winding1=[ trans(10,4)*1e3, 1e-6 , 0 ]  Winding2=[ trans(10,5)*1e3, 0 , trans(10,7) ]  Rm=500  Lm=500  L0=0.5  Saturation=[ 0,0 ; 0.0024,1.2 ; 1.0,1.52 ]  InitialFluxes=[ 0.8 , -0.8 , 0.7 ]  MoreParameters=off  BreakLoop=off  DataType=off  TransfoNumber=0
  T102 : powerlib/Elements/Three-Phase Transformer (Two Windings)  Winding1Connection=Yg  Winding2Connection=Yg  CoreType=Three single-phase transformers  SetSaturation=off  Hysteresis=off  DataFile='hysteresis'  SetInitialFlux=off  Measurements=None  UNITS=pu  NominalPower=[ trans(1,6)*1e6 , 50 ]  Winding1=[ trans(1,4)*1e3, 1e-6, 0 ]  Winding2=[ trans(1,5)*1e3, 1e-6, trans(1,7) ]  Rm=500  Lm=500  L0=0.5  Saturation=[ 0,0 ; 0.0024,1.2 ; 1.0,1.52 ]  InitialFluxes=[ 0.8 , -0.8 , 0.7 ]  MoreParameters=off  BreakLoop=off  DataType=off  TransfoNumber=0
  T11 : powerlib/Elements/Three-Phase Transformer (Two Windings)  Winding1Connection=Y  Winding2Connection=Y  CoreType=Three single-phase transformers  SetSaturation=off  Hysteresis=off  DataFile='hysteresis'  SetInitialFlux=off  Measurements=None  UNITS=pu  NominalPower=[ trans(11,6)*1e6 , 50 ]  Winding1=[ trans(11,4)*1e3, 1e-6, 0 ]  Winding2=[ trans(11,5)*1e3, 0 , trans(11,7) ]  Rm=500  Lm=500  L0=0.5  Saturation=[ 0,0 ; 0.0024,1.2 ; 1.0,1.52 ]  InitialFluxes=[ 0.8 , -0.8 , 0.7 ]  MoreParameters=off  BreakLoop=off  DataType=off  TransfoNumber=0
  T12 : powerlib/Elements/Three-Phase Transformer (Two Windings)  Winding1Connection=Y  Winding2Connection=Y  CoreType=Three single-phase transformers  SetSaturation=off  Hysteresis=off  DataFile='hysteresis'  SetInitialFlux=off  Measurements=None  UNITS=pu  NominalPower=[ trans(12,6)*1e6 , 50 ]  Winding1=[ trans(12,4)*1e3, 1e-6, 0 ]  Winding2=[ trans(12,5)*1e3, 0 , trans(12,7)]  Rm=500  Lm=500  L0=0.5  Saturation=[ 0,0 ; 0.0024,1.2 ; 1.0,1.52 ]  InitialFluxes=[ 0.8 , -0.8 , 0.7 ]  MoreParameters=off  BreakLoop=off  DataType=off  TransfoNumber=0
  T13 : powerlib/Elements/Three-Phase Transformer (Two Windings)  Winding1Connection=Y  Winding2Connection=Y  CoreType=Three single-phase transformers  SetSaturation=off  Hysteresis=off  DataFile='hysteresis'  SetInitialFlux=off  Measurements=None  UNITS=pu  NominalPower=[ trans(13,6)*1e6 , 50 ]  Winding1=[ trans(13,4)*1e3, 1e-6, 0 ]  Winding2=[ trans(13,5)*1e3, 0 , trans(13,7) ]  Rm=500  Lm=500  L0=0.5  Saturation=[ 0,0 ; 0.0024,1.2 ; 1.0,1.52 ]  InitialFluxes=[ 0.8 , -0.8 , 0.7 ]  MoreParameters=off  BreakLoop=off  DataType=off  TransfoNumber=0
  T14 : powerlib/Elements/Three-Phase Transformer (Two Windings)  Winding1Connection=Delta (D1)  Winding2Connection=Yg  CoreType=Three single-phase transformers  SetSaturation=off  Hysteresis=off  DataFile='hysteresis'  SetInitialFlux=off  Measurements=None  UNITS=pu  NominalPower=[ trans(14,6)*1e6 , 50 ]  Winding1=[ trans(14,4)*1e3, 1e-6 , 0 ]  Winding2=[ trans(14,5)*1e3, 0 , trans(14,7) ]  Rm=500  Lm=500  L0=0.5  Saturation=[ 0,0 ; 0.0024,1.2 ; 1.0,1.52 ]  InitialFluxes=[ 0.8 , -0.8 , 0.7 ]  MoreParameters=off  BreakLoop=off  DataType=off  TransfoNumber=0
  T15 : powerlib/Elements/Three-Phase Transformer (Two Windings)  Winding1Connection=Yg  Winding2Connection=Yg  CoreType=Three single-phase transformers  SetSaturation=off  Hysteresis=off  DataFile='hysteresis'  SetInitialFlux=off  Measurements=None  UNITS=pu  NominalPower=[ trans(15,6)*1e6 , 50 ]  Winding1=[ trans(15,4)*1e3, 1e-6 , 0 ]  Winding2=[ trans(15,5)*1e3, 0 , trans(15,7) ]  Rm=500  Lm=500  L0=0.5  Saturation=[ 0,0 ; 0.0024,1.2 ; 1.0,1.52 ]  InitialFluxes=[ 0.8 , -0.8 , 0.7 ]  MoreParameters=off  BreakLoop=off  DataType=off  TransfoNumber=0
  T16 : powerlib/Elements/Three-Phase Transformer (Two Windings)  Winding1Connection=Yg  Winding2Connection=Yg  CoreType=Three single-phase transformers  SetSaturation=off  Hysteresis=off  DataFile='hysteresis'  SetInitialFlux=off  Measurements=None  UNITS=pu  NominalPower=[ trans(16,6)*1e6 , 50 ]  Winding1=[ trans(16,4)*1e3, 1e-6 , 0]  Winding2=[ trans(16,5)*1e3, 0 , trans(16,7) ]  Rm=500  Lm=500  L0=0.5  Saturation=[ 0,0 ; 0.0024,1.2 ; 1.0,1.52 ]  InitialFluxes=[ 0.8 , -0.8 , 0.7 ]  MoreParameters=off  BreakLoop=off  DataType=off  TransfoNumber=0
  T17 : powerlib/Elements/Three-Phase Transformer (Two Windings)  Winding1Connection=Delta (D1)  Winding2Connection=Yg  CoreType=Three single-phase transformers  SetSaturation=off  Hysteresis=off  DataFile='hysteresis'  SetInitialFlux=off  Measurements=None  UNITS=pu  NominalPower=[ trans(17,6)*1e6 , 50 ]  Winding1=[ trans(17,4)*1e3, 1e-6 , 0 ]  Winding2=[ trans(17,5)*1e3, 0 , trans(17,7) ]  Rm=500  Lm=500  L0=0.5  Saturation=[ 0,0 ; 0.0024,1.2 ; 1.0,1.52 ]  InitialFluxes=[ 0.8 , -0.8 , 0.7 ]  MoreParameters=off  BreakLoop=off  DataType=off  TransfoNumber=0
  T18-1 : powerlib/Elements/Three-Phase Transformer (Two Windings)  Winding1Connection=Y  Winding2Connection=Y  CoreType=Three single-phase transformers  SetSaturation=off  Hysteresis=off  DataFile='hysteresis'  SetInitialFlux=off  Measurements=None  UNITS=pu  NominalPower=[ trans(18,6)*1e6 , 50 ]  Winding1=[ trans(18,4)*1e3, 1e-6, 0 ]  Winding2=[ trans(18,5)*1e3, 0 , trans(18,7) ]  Rm=500  Lm=500  L0=0.5  Saturation=[ 0,0 ; 0.0024,1.2 ; 1.0,1.52 ]  InitialFluxes=[ 0.8 , -0.8 , 0.7 ]  MoreParameters=off  BreakLoop=off  DataType=off  TransfoNumber=0
  T18-2 : powerlib/Elements/Three-Phase Transformer (Two Windings)  Winding1Connection=Y  Winding2Connection=Y  CoreType=Three single-phase transformers  SetSaturation=off  Hysteresis=off  DataFile='hysteresis'  SetInitialFlux=off  Measurements=None  UNITS=pu  NominalPower=[ trans(18,6)*1e6 , 50 ]  Winding1=[ trans(18,4)*1e3, 1e-6, 0 ]  Winding2=[ trans(18,5)*1e3, 0 , trans(18,7) ]  Rm=500  Lm=500  L0=0.5  Saturation=[ 0,0 ; 0.0024,1.2 ; 1.0,1.52 ]  InitialFluxes=[ 0.8 , -0.8 , 0.7 ]  MoreParameters=off  BreakLoop=off  DataType=off  TransfoNumber=0
  T19 : powerlib/Elements/Three-Phase Transformer (Two Windings)  Winding1Connection=Delta (D1)  Winding2Connection=Yg  CoreType=Three single-phase transformers  SetSaturation=off  Hysteresis=off  DataFile='hysteresis'  SetInitialFlux=off  Measurements=None  UNITS=pu  NominalPower=[ trans(19,6)*1e6 , 50 ]  Winding1=[ trans(19,4)*1e3, 1e-6 , 0 ]  Winding2=[ trans(19,5)*1e3, 0 , trans(19,7) ]  Rm=500  Lm=500  L0=0.5  Saturation=[ 0,0 ; 0.0024,1.2 ; 1.0,1.52 ]  InitialFluxes=[ 0.8 , -0.8 , 0.7 ]  MoreParameters=off  BreakLoop=off  DataType=off  TransfoNumber=0
  T2 : powerlib/Elements/Three-Phase Transformer (Two Windings)  Winding1Connection=Delta (D1)  Winding2Connection=Yg  CoreType=Three single-phase transformers  SetSaturation=off  Hysteresis=off  DataFile='hysteresis'  SetInitialFlux=off  Measurements=None  UNITS=pu  NominalPower=[ trans(2,6)*1e6 , 50 ]  Winding1=[ trans(2,4)*1e3, 1e-6 , 0 ]  Winding2=[ trans(2,5)*1e3, 0 , trans(2,7) ]  Rm=500  Lm=500  L0=0.5  Saturation=[ 0,0 ; 0.0024,1.2 ; 1.0,1.52 ]  InitialFluxes=[ 0.8 , -0.8 , 0.7 ]  MoreParameters=off  BreakLoop=off  DataType=off  TransfoNumber=0
  T20 : powerlib/Elements/Three-Phase Transformer (Two Windings)  Winding1Connection=Yg  Winding2Connection=Yg  CoreType=Three single-phase transformers  SetSaturation=off  Hysteresis=off  DataFile='hysteresis'  SetInitialFlux=off  Measurements=None  UNITS=pu  NominalPower=[ trans(20,6)*1e6 , 50 ]  Winding1=[ trans(20,4)*1e3, 1e-6 , 0]  Winding2=[ trans(20,5)*1e3, 0 , trans(20,7) ]  Rm=500  Lm=500  L0=0.5  Saturation=[ 0,0 ; 0.0024,1.2 ; 1.0,1.52 ]  InitialFluxes=[ 0.8 , -0.8 , 0.7 ]  MoreParameters=off  BreakLoop=off  DataType=off  TransfoNumber=0
  T208 : powerlib/Elements/Three-Phase Transformer (Two Windings)  Winding1Connection=Yg  Winding2Connection=Yg  CoreType=Three single-phase transformers  SetSaturation=off  Hysteresis=off  DataFile='hysteresis'  SetInitialFlux=off  Measurements=None  UNITS=pu  NominalPower=[ trans(4,6)*1e6 , 50 ]  Winding1=[ trans(4,4)*1e3, 1e-6 , 0 ]  Winding2=[ trans(4,5)*1e3, 0 , trans(4,7) ]  Rm=500  Lm=500  L0=0.5  Saturation=[ 0,0 ; 0.0024,1.2 ; 1.0,1.52 ]  InitialFluxes=[ 0.8 , -0.8 , 0.7 ]  MoreParameters=off  BreakLoop=off  DataType=off  TransfoNumber=0
  T21 : powerlib/Elements/Three-Phase Transformer (Two Windings)  Winding1Connection=Delta (D1)  Winding2Connection=Yg  CoreType=Three single-phase transformers  SetSaturation=off  Hysteresis=off  DataFile='hysteresis'  SetInitialFlux=off  Measurements=None  UNITS=pu  NominalPower=[ trans(21,6)*1e6 , 50 ]  Winding1=[ trans(21,4)*1e3, 1e-6 , 0 ]  Winding2=[ trans(21,5)*1e3, 0 , trans(21,7) ]  Rm=500  Lm=500  L0=0.5  Saturation=[ 0,0 ; 0.0024,1.2 ; 1.0,1.52 ]  InitialFluxes=[ 0.8 , -0.8 , 0.7 ]  MoreParameters=off  BreakLoop=off  DataType=off  TransfoNumber=0
  T212 : powerlib/Elements/Three-Phase Transformer (Two Windings)  Winding1Connection=Yg  Winding2Connection=Yg  CoreType=Three single-phase transformers  SetSaturation=off  Hysteresis=off  DataFile='hysteresis'  SetInitialFlux=off  Measurements=None  UNITS=pu  NominalPower=[ trans(4,6)*1e6 , 50 ]  Winding1=[ trans(4,4)*1e3, 1e-6 , 0 ]  Winding2=[ trans(4,5)*1e3, 0 , trans(4,7) ]  Rm=500  Lm=500  L0=0.5  Saturation=[ 0,0 ; 0.0024,1.2 ; 1.0,1.52 ]  InitialFluxes=[ 0.8 , -0.8 , 0.7 ]  MoreParameters=off  BreakLoop=off  DataType=off  TransfoNumber=0
  T215 : powerlib/Elements/Three-Phase Transformer (Two Windings)  Winding1Connection=Yg  Winding2Connection=Yg  CoreType=Three single-phase transformers  SetSaturation=off  Hysteresis=off  DataFile='hysteresis'  SetInitialFlux=off  Measurements=None  UNITS=pu  NominalPower=[ trans(5,6)*1e6 , 50 ]  Winding1=[ trans(5,4)*1e3, 1e-6 , 0 ]  Winding2=[ trans(5,5)*1e3, 0 , trans(5,7) ]  Rm=500  Lm=500  L0=0.5  Saturation=[ 0,0 ; 0.0024,1.2 ; 1.0,1.52 ]  InitialFluxes=[ 0.8 , -0.8 , 0.7 ]  MoreParameters=off  BreakLoop=off  DataType=off  TransfoNumber=0
  T216 : powerlib/Elements/Three-Phase Transformer (Two Windings)  Winding1Connection=Yg  Winding2Connection=Yg  CoreType=Three single-phase transformers  SetSaturation=off  Hysteresis=off  DataFile='hysteresis'  SetInitialFlux=off  Measurements=None  UNITS=pu  NominalPower=[ trans(5,6)*1e6 , 50 ]  Winding1=[ trans(5,4)*1e3, 1e-6 , 0 ]  Winding2=[ trans(5,5)*1e3, 0 , trans(5,7) ]  Rm=500  Lm=500  L0=0.5  Saturation=[ 0,0 ; 0.0024,1.2 ; 1.0,1.52 ]  InitialFluxes=[ 0.8 , -0.8 , 0.7 ]  MoreParameters=off  BreakLoop=off  DataType=off  TransfoNumber=0
  T3 : powerlib/Elements/Three-Phase Transformer (Two Windings)  Winding1Connection=Delta (D1)  Winding2Connection=Yg  CoreType=Three single-phase transformers  SetSaturation=off  Hysteresis=off  DataFile='hysteresis'  SetInitialFlux=off  Measurements=None  UNITS=pu  NominalPower=[ trans(3,6)*1e6 , 50 ]  Winding1=[ trans(3,4)*1e3, 1e-6 , 0 ]  Winding2=[ trans(3,5)*1e3, 0 , trans(3,7) ]  Rm=500  Lm=500  L0=0.5  Saturation=[ 0,0 ; 0.0024,1.2 ; 1.0,1.52 ]  InitialFluxes=[ 0.8 , -0.8 , 0.7 ]  MoreParameters=off  BreakLoop=off  DataType=off  TransfoNumber=0
  T308 : powerlib/Elements/Three-Phase Transformer (Two Windings)  Winding1Connection=Yg  Winding2Connection=Yg  CoreType=Three single-phase transformers  SetSaturation=off  Hysteresis=off  DataFile='hysteresis'  SetInitialFlux=off  Measurements=None  UNITS=pu  NominalPower=[ trans(8,6)*1e6 , 50 ]  Winding1=[ trans(8,4)*1e3, 1e-6 , 0 ]  Winding2=[ trans(8,5)*1e3, 0 , trans(8,7)]  Rm=500  Lm=500  L0=0.5  Saturation=[ 0,0 ; 0.0024,1.2 ; 1.0,1.52 ]  InitialFluxes=[ 0.8 , -0.8 , 0.7 ]  MoreParameters=off  BreakLoop=off  DataType=off  TransfoNumber=0
  T309 : powerlib/Elements/Three-Phase Transformer (Two Windings)  Winding1Connection=Yg  Winding2Connection=Yg  CoreType=Three single-phase transformers  SetSaturation=off  Hysteresis=off  DataFile='hysteresis'  SetInitialFlux=off  Measurements=None  UNITS=pu  NominalPower=[ trans(1,6)*1e6 , 50 ]  Winding1=[ trans(1,4)*1e3, 1e-6, 0 ]  Winding2=[ trans(1,5)*1e3, 1e-6, trans(1,7) ]  Rm=500  Lm=500  L0=0.5  Saturation=[ 0,0 ; 0.0024,1.2 ; 1.0,1.52 ]  InitialFluxes=[ 0.8 , -0.8 , 0.7 ]  MoreParameters=off  BreakLoop=off  DataType=off  TransfoNumber=0
  T312 : powerlib/Elements/Three-Phase Transformer (Two Windings)  Winding1Connection=Yg  Winding2Connection=Yg  CoreType=Three single-phase transformers  SetSaturation=off  Hysteresis=off  DataFile='hysteresis'  SetInitialFlux=off  Measurements=None  UNITS=pu  NominalPower=[ trans(9,6)*1e6 , 50 ]  Winding1=[ trans(9,4)*1e3, 1e-6, 0 ]  Winding2=[ trans(9,5)*1e3, 0 , trans(9,7)]  Rm=500  Lm=500  L0=0.5  Saturation=[ 0,0 ; 0.0024,1.2 ; 1.0,1.52 ]  InitialFluxes=[ 0.8 , -0.8 , 0.7 ]  MoreParameters=off  BreakLoop=off  DataType=off  TransfoNumber=0
  T314 : powerlib/Elements/Three-Phase Transformer (Two Windings)  Winding1Connection=Yg  Winding2Connection=Yg  CoreType=Three single-phase transformers  SetSaturation=off  Hysteresis=off  DataFile='hysteresis'  SetInitialFlux=off  Measurements=None  UNITS=pu  NominalPower=[ trans(9,6)*1e6 , 50 ]  Winding1=[ trans(9,4)*1e3, 1e-6, 0 ]  Winding2=[ trans(9,5)*1e3, 0 , trans(9,7)]  Rm=500  Lm=500  L0=0.5  Saturation=[ 0,0 ; 0.0024,1.2 ; 1.0,1.52 ]  InitialFluxes=[ 0.8 , -0.8 , 0.7 ]  MoreParameters=off  BreakLoop=off  DataType=off  TransfoNumber=0
  T35 : powerlib/Elements/Three-Phase Transformer (Two Windings)  Winding1Connection=Yg  Winding2Connection=Yg  CoreType=Three single-phase transformers  SetSaturation=off  Hysteresis=off  DataFile='hysteresis'  SetInitialFlux=off  Measurements=None  UNITS=pu  NominalPower=[ trans(14,6)*1e6 , 50 ]  Winding1=[ trans(14,4)*1e3, 1e-6 , 0 ]  Winding2=[ trans(14,5)*1e3, 0 , trans(14,7) ]  Rm=500  Lm=500  L0=0.5  Saturation=[ 0,0 ; 0.0024,1.2 ; 1.0,1.52 ]  InitialFluxes=[ 0.8 , -0.8 , 0.7 ]  MoreParameters=off  BreakLoop=off  DataType=off  TransfoNumber=0
  T36 : powerlib/Elements/Three-Phase Transformer (Two Windings)  Winding1Connection=Yg  Winding2Connection=Yg  CoreType=Three single-phase transformers  SetSaturation=off  Hysteresis=off  DataFile='hysteresis'  SetInitialFlux=off  Measurements=None  UNITS=pu  NominalPower=[ trans(14,6)*1e6 , 50 ]  Winding1=[ trans(14,4)*1e3, 1e-6 , 0 ]  Winding2=[ trans(14,5)*1e3, 0 , trans(14,7) ]  Rm=500  Lm=500  L0=0.5  Saturation=[ 0,0 ; 0.0024,1.2 ; 1.0,1.52 ]  InitialFluxes=[ 0.8 , -0.8 , 0.7 ]  MoreParameters=off  BreakLoop=off  DataType=off  TransfoNumber=0
  T37 : powerlib/Elements/Three-Phase Transformer (Two Windings)  Winding1Connection=Yg  Winding2Connection=Yg  CoreType=Three single-phase transformers  SetSaturation=off  Hysteresis=off  DataFile='hysteresis'  SetInitialFlux=off  Measurements=None  UNITS=pu  NominalPower=[ trans(2,6)*1e6 , 50 ]  Winding1=[ trans(2,4)*1e3, 1e-6 , 0 ]  Winding2=[ trans(2,5)*1e3, 0 , trans(2,7) ]  Rm=500  Lm=500  L0=0.5  Saturation=[ 0,0 ; 0.0024,1.2 ; 1.0,1.52 ]  InitialFluxes=[ 0.8 , -0.8 , 0.7 ]  MoreParameters=off  BreakLoop=off  DataType=off  TransfoNumber=0
  T38 : powerlib/Elements/Three-Phase Transformer (Two Windings)  Winding1Connection=Yg  Winding2Connection=Yg  CoreType=Three single-phase transformers  SetSaturation=off  Hysteresis=off  DataFile='hysteresis'  SetInitialFlux=off  Measurements=None  UNITS=pu  NominalPower=[ trans(4,6)*1e6 , 50 ]  Winding1=[ trans(4,4)*1e3, 1e-6 , 0 ]  Winding2=[ trans(4,5)*1e3, 0 , trans(4,7) ]  Rm=500  Lm=500  L0=0.5  Saturation=[ 0,0 ; 0.0024,1.2 ; 1.0,1.52 ]  InitialFluxes=[ 0.8 , -0.8 , 0.7 ]  MoreParameters=off  BreakLoop=off  DataType=off  TransfoNumber=0
  T39 : powerlib/Elements/Three-Phase Transformer (Two Windings)  Winding1Connection=Yg  Winding2Connection=Yg  CoreType=Three single-phase transformers  SetSaturation=off  Hysteresis=off  DataFile='hysteresis'  SetInitialFlux=off  Measurements=None  UNITS=pu  NominalPower=[ trans(8,6)*1e6 , 50 ]  Winding1=[ trans(8,4)*1e3, 1e-6 , 0 ]  Winding2=[ trans(8,5)*1e3, 0 , trans(8,7)]  Rm=500  Lm=500  L0=0.5  Saturation=[ 0,0 ; 0.0024,1.2 ; 1.0,1.52 ]  InitialFluxes=[ 0.8 , -0.8 , 0.7 ]  MoreParameters=off  BreakLoop=off  DataType=off  TransfoNumber=0
  T4 : powerlib/Elements/Three-Phase Transformer (Two Windings)  Winding1Connection=Delta (D1)  Winding2Connection=Yg  CoreType=Three single-phase transformers  SetSaturation=off  Hysteresis=off  DataFile='hysteresis'  SetInitialFlux=off  Measurements=None  UNITS=pu  NominalPower=[ trans(4,6)*1e6 , 50 ]  Winding1=[ trans(4,4)*1e3, 1e-6 , 0 ]  Winding2=[ trans(4,5)*1e3, 0 , trans(4,7) ]  Rm=500  Lm=500  L0=0.5  Saturation=[ 0,0 ; 0.0024,1.2 ; 1.0,1.52 ]  InitialFluxes=[ 0.8 , -0.8 , 0.7 ]  MoreParameters=off  BreakLoop=off  DataType=off  TransfoNumber=0
  T40 : powerlib/Elements/Three-Phase Transformer (Two Windings)  Winding1Connection=Yg  Winding2Connection=Yg  CoreType=Three single-phase transformers  SetSaturation=off  Hysteresis=off  DataFile='hysteresis'  SetInitialFlux=off  Measurements=None  UNITS=pu  NominalPower=[ trans(21,6)*1e6 , 50 ]  Winding1=[ trans(21,4)*1e3, 1e-6 , 0 ]  Winding2=[ trans(21,5)*1e3, 0 , trans(21,7) ]  Rm=500  Lm=500  L0=0.5  Saturation=[ 0,0 ; 0.0024,1.2 ; 1.0,1.52 ]  InitialFluxes=[ 0.8 , -0.8 , 0.7 ]  MoreParameters=off  BreakLoop=off  DataType=off  TransfoNumber=0
  T405 : powerlib/Elements/Three-Phase Transformer (Two Windings)  Winding1Connection=Yg  Winding2Connection=Yg  CoreType=Three single-phase transformers  SetSaturation=off  Hysteresis=off  DataFile='hysteresis'  SetInitialFlux=off  Measurements=None  UNITS=pu  NominalPower=[ trans(17,6)*1e6 , 50 ]  Winding1=[ trans(17,4)*1e3, 1e-6 , 0 ]  Winding2=[ trans(17,5)*1e3, 0 , trans(17,7) ]  Rm=500  Lm=500  L0=0.5  Saturation=[ 0,0 ; 0.0024,1.2 ; 1.0,1.52 ]  InitialFluxes=[ 0.8 , -0.8 , 0.7 ]  MoreParameters=off  BreakLoop=off  DataType=off  TransfoNumber=0
  T410 : powerlib/Elements/Three-Phase Transformer (Two Windings)  Winding1Connection=Yg  Winding2Connection=Yg  CoreType=Three single-phase transformers  SetSaturation=off  Hysteresis=off  DataFile='hysteresis'  SetInitialFlux=off  Measurements=None  UNITS=pu  NominalPower=[ trans(14,6)*1e6 , 50 ]  Winding1=[ trans(14,4)*1e3, 1e-6 , 0 ]  Winding2=[ trans(14,5)*1e3, 0 , trans(14,7) ]  Rm=500  Lm=500  L0=0.5  Saturation=[ 0,0 ; 0.0024,1.2 ; 1.0,1.52 ]  InitialFluxes=[ 0.8 , -0.8 , 0.7 ]  MoreParameters=off  BreakLoop=off  DataType=off  TransfoNumber=0
  T5 : powerlib/Elements/Three-Phase Transformer (Two Windings)  Winding1Connection=Delta (D1)  Winding2Connection=Yg  CoreType=Three single-phase transformers  SetSaturation=off  Hysteresis=off  DataFile='hysteresis'  SetInitialFlux=off  Measurements=None  UNITS=pu  NominalPower=[ trans(5,6)*1e6 , 50 ]  Winding1=[ trans(5,4)*1e3, 1e-6 , 0 ]  Winding2=[ trans(5,5)*1e3, 0 , trans(5,7) ]  Rm=500  Lm=500  L0=0.5  Saturation=[ 0,0 ; 0.0024,1.2 ; 1.0,1.52 ]  InitialFluxes=[ 0.8 , -0.8 , 0.7 ]  MoreParameters=off  BreakLoop=off  DataType=off  TransfoNumber=0
  T502 : powerlib/Elements/Three-Phase Transformer (Two Windings)  Winding1Connection=Yg  Winding2Connection=Yg  CoreType=Three single-phase transformers  SetSaturation=off  Hysteresis=off  DataFile='hysteresis'  SetInitialFlux=off  Measurements=None  UNITS=pu  NominalPower=[ trans(19,6)*1e6 , 50 ]  Winding1=[ trans(19,4)*1e3, 1e-6 , 0 ]  Winding2=[ trans(19,5)*1e3, 0 , trans(19,7) ]  Rm=500  Lm=500  L0=0.5  Saturation=[ 0,0 ; 0.0024,1.2 ; 1.0,1.52 ]  InitialFluxes=[ 0.8 , -0.8 , 0.7 ]  MoreParameters=off  BreakLoop=off  DataType=off  TransfoNumber=0
  T504 : powerlib/Elements/Three-Phase Transformer (Two Windings)  Winding1Connection=Yg  Winding2Connection=Yg  CoreType=Three single-phase transformers  SetSaturation=off  Hysteresis=off  DataFile='hysteresis'  SetInitialFlux=off  Measurements=None  UNITS=pu  NominalPower=[ trans(19,6)*1e6 , 50 ]  Winding1=[ trans(19,4)*1e3, 1e-6 , 0 ]  Winding2=[ trans(19,5)*1e3, 0 , trans(19,7) ]  Rm=500  Lm=500  L0=0.5  Saturation=[ 0,0 ; 0.0024,1.2 ; 1.0,1.52 ]  InitialFluxes=[ 0.8 , -0.8 , 0.7 ]  MoreParameters=off  BreakLoop=off  DataType=off  TransfoNumber=0
  T508 : powerlib/Elements/Three-Phase Transformer (Two Windings)  Winding1Connection=Yg  Winding2Connection=Yg  CoreType=Three single-phase transformers  SetSaturation=off  Hysteresis=off  DataFile='hysteresis'  SetInitialFlux=off  Measurements=None  UNITS=pu  NominalPower=[ trans(21,6)*1e6 , 50 ]  Winding1=[ trans(21,4)*1e3, 1e-6 , 0 ]  Winding2=[ trans(21,5)*1e3, 0 , trans(21,7) ]  Rm=500  Lm=500  L0=0.5  Saturation=[ 0,0 ; 0.0024,1.2 ; 1.0,1.52 ]  InitialFluxes=[ 0.8 , -0.8 , 0.7 ]  MoreParameters=off  BreakLoop=off  DataType=off  TransfoNumber=0
  T6 : powerlib/Elements/Three-Phase Transformer (Two Windings)  Winding1Connection=Y  Winding2Connection=Y  CoreType=Three single-phase transformers  SetSaturation=off  Hysteresis=off  DataFile='hysteresis'  SetInitialFlux=off  Measurements=None  UNITS=pu  NominalPower=[ trans(6,6)*1e6 , 50 ]  Winding1="[ trans(6,4)*1e3, 1e-6, 0  ]"  Winding2=[ trans(6,5)*1e3, 0 , trans(6,7)]  Rm=500  Lm=500  L0=0.5  Saturation=[ 0,0 ; 0.0024,1.2 ; 1.0,1.52 ]  InitialFluxes=[ 0.8 , -0.8 , 0.7 ]  MoreParameters=off  BreakLoop=off  DataType=off  TransfoNumber=0
  T7 : powerlib/Elements/Three-Phase Transformer (Two Windings)  Winding1Connection=Y  Winding2Connection=Y  CoreType=Three single-phase transformers  SetSaturation=off  Hysteresis=off  DataFile='hysteresis'  SetInitialFlux=off  Measurements=None  UNITS=pu  NominalPower=[ trans(7,6)*1e6 , 50 ]  Winding1=[ trans(7,4)*1e3, 1e-6, 0 ]  Winding2=[ trans(7,5)*1e3, 0 , trans(7,7) ]  Rm=500  Lm=500  L0=0.5  Saturation=[ 0,0 ; 0.0024,1.2 ; 1.0,1.52 ]  InitialFluxes=[ 0.8 , -0.8 , 0.7 ]  MoreParameters=off  BreakLoop=off  DataType=off  TransfoNumber=0
  T8 : powerlib/Elements/Three-Phase Transformer (Two Windings)  Winding1Connection=Delta (D1)  Winding2Connection=Yg  CoreType=Three single-phase transformers  SetSaturation=off  Hysteresis=off  DataFile='hysteresis'  SetInitialFlux=off  Measurements=None  UNITS=pu  NominalPower=[ trans(8,6)*1e6 , 50 ]  Winding1=[ trans(8,4)*1e3, 1e-6 , 0 ]  Winding2=[ trans(8,5)*1e3, 0 , trans(8,7)]  Rm=500  Lm=500  L0=0.5  Saturation=[ 0,0 ; 0.0024,1.2 ; 1.0,1.52 ]  InitialFluxes=[ 0.8 , -0.8 , 0.7 ]  MoreParameters=off  BreakLoop=off  DataType=off  TransfoNumber=0
  T9 : powerlib/Elements/Three-Phase Transformer (Two Windings)  Winding1Connection=Delta (D1)  Winding2Connection=Yg  CoreType=Three single-phase transformers  SetSaturation=off  Hysteresis=off  DataFile='hysteresis'  SetInitialFlux=off  Measurements=None  UNITS=pu  NominalPower=[ trans(9,6)*1e6 , 50 ]  Winding1=[ trans(9,4)*1e3, 1e-6, 0 ]  Winding2=[ trans(9,5)*1e3, 0 , trans(9,7)]  Rm=500  Lm=500  L0=0.5  Saturation=[ 0,0 ; 0.0024,1.2 ; 1.0,1.52 ]  InitialFluxes=[ 0.8 , -0.8 , 0.7 ]  MoreParameters=off  BreakLoop=off  DataType=off  TransfoNumber=0
  Three-Phase V-I Measurement{1..4} (4 alike) : powerlib/Measurements/Three-Phase V-I Measurement  VoltageMeasurement=phase-to-ground  SetLabelV=off  LabelV=Vabc  Vpu=off  VpuLL=off  CurrentMeasurement=yes  SetLabelI=off  LabelI=Iabc  Ipu=off  Pbase=100e6  Vbase=500e3  OutputType=Complex  PhasorSimulation=on  PSBequivalent=0
  Three-Phase Breaker : powerlib/Elements/Three-Phase Breaker  InitialState=closed  SwitchA=on  SwitchB=on  SwitchC=on  SwitchTimes=dist.tsplit  External=off  BreakerResistance=0.01  SnubberResistance=1e6  SnubberCapacitance=inf  Measurements=None
  Three-Phase Breaker1 : powerlib/Elements/Three-Phase Breaker  InitialState=closed  SwitchA=on  SwitchB=on  SwitchC=on  SwitchTimes=dist.tgen  External=off  BreakerResistance=0.01  SnubberResistance=1e6  SnubberCapacitance=inf  Measurements=None
  Three-Phase Breaker2 : powerlib/Elements/Three-Phase Breaker  Commented=on  InitialState=open  SwitchA=on  SwitchB=on  SwitchC=on  SwitchTimes=dist.tgen  External=off  BreakerResistance=0.01  SnubberResistance=1e6  SnubberCapacitance=inf  Measurements=None
  VI102 : Subsystem
  VI102_form : Subsystem  Commented=on
  VI208 : Subsystem
  VI208_form : Subsystem  Commented=on
  VI212 : Subsystem
  VI212_form : Subsystem  Commented=on
  VI215 : Subsystem
  VI215_form : Subsystem  Commented=on
  VI216 : Subsystem
  VI216_form : Subsystem  Commented=on
  VI308 : Subsystem
  VI308_form : Subsystem  Commented=on
  VI309 : Subsystem
  VI309_form : Subsystem  Commented=on
  VI312 : Subsystem
  VI312_form : Subsystem  Commented=on
  VI314 : Subsystem
  VI314_form : Subsystem  Commented=on
  VI403 : Subsystem
  VI403_form : Subsystem  Commented=on
  VI405 : Subsystem
  VI405_form : Subsystem  Commented=on
  VI410 : Subsystem
  VI410_form : Subsystem  Commented=on
  VI502 : Subsystem
  VI502_form : Subsystem  Commented=on
  VI504 : Subsystem
  VI504_form : Subsystem  Commented=on
  VI508 : Subsystem
  VI508_form : Subsystem  Commented=on
  Voltage Measurement : powerlib/Measurements/Voltage Measurement  PhasorSimulation=on  OutputType=Magnitude  PSBequivalent=0
  powergui : powerlib/powergui  Priority=1  SimulationMode=Phasor  SampleTime=50e-6  frequency=50  Iterations=50  frequencyindice=50  Pbase=100e6  ErrMax=0.0001  UnitsV=kV  UnitsW=MW  buscounter=0  FunctionMessages=off  echomessages=off  EnableUseOfTLC=off  CurrentSourceSwitches=off  DisableSnubberDevices=off  DisableRonSwitches=off  DisableVfSwitches=off  DisplayEquations=off  SolverType=Tustin  Interpol=off  ExternalGateDelay=off  methode=off  Ts=100  x0status=blocks  SPID=off  SwTol=0  HookPort=off  RestoreLinks=warning  ResistiveCurrentMeasurement=off  Frange=[0:2:500]  Ylog=off  Xlog=on  ShowGrid=off  save=off  variable=ZData  structure=0  ZoomFFT=off  StartTime=0.0  cycles=1  DisplayStyle=1  fundamental=60  FreqAxis=off  MaxFrequency=1000  frequencyindicesteady=1  RmsSteady=1  display=off
  tag scope: PSSmodel=global
  wires:
  Demux/1 -> P 4-2/1
  Demux/2 -> P 4-2/2
  3-Phase Active & Reactive Power (Phasor Type)1/1 -> Demux/1
  Three-Phase V-I Measurement1/2 -> 3-Phase Active & Reactive Power (Phasor Type)1/2
  Three-Phase V-I Measurement1/1 -> 3-Phase Active & Reactive Power (Phasor Type)1/1
  Demux1/1 -> P 2-1/1
  Three-Phase V-I Measurement2/2 -> 3-Phase Active & Reactive Power (Phasor Type)2/2
  Three-Phase V-I Measurement2/1 -> 3-Phase Active & Reactive Power (Phasor Type)2/1
  3-Phase Active & Reactive Power (Phasor Type)2/1 -> Demux1/1
  Demux1/2 -> P 2-1/2
  Demux2/1 -> P 1-3/1
  3-Phase Active & Reactive Power (Phasor Type)3/1 -> Demux2/1
  Demux2/2 -> P 1-3/2
  Three-Phase V-I Measurement3/1 -> 3-Phase Active & Reactive Power (Phasor Type)3/1
  Three-Phase V-I Measurement3/2 -> 3-Phase Active & Reactive Power (Phasor Type)3/2
  Demux3/1 -> P 3-5/1
  3-Phase Active & Reactive Power (Phasor Type)4/1 -> Demux3/1
  Demux3/2 -> P 3-5/2
  Three-Phase V-I Measurement4/2 -> 3-Phase Active & Reactive Power (Phasor Type)4/2
  Three-Phase V-I Measurement4/1 -> 3-Phase Active & Reactive Power (Phasor Type)4/1
  PSS model/1 -> [PSSmodel]
  Voltage Measurement/1 -> Scope/1
  connections:
  L-38-1/LConn1 -- L-35-1/LConn1 -- L-35-2/LConn1 -- B406/RConn1 -- L-38-2/LConn1
  B406/RConn2 -- L-35-1/LConn2 -- L-35-2/LConn2 -- L-38-1/LConn2 -- L-38-2/LConn2
  L-35-1/LConn3 -- L-35-2/LConn3 -- B406/RConn3 -- L-38-1/LConn3 -- L-38-2/LConn3
  B407/RConn1 -- L-38-1/RConn1 -- L-38-2/RConn1
  B407/RConn2 -- L-38-1/RConn2 -- L-38-2/RConn2
  B407/RConn3 -- L-38-1/RConn3 -- L-38-2/RConn3
  B405/RConn1 -- L-35-2/RConn1 -- L-35-1/RConn1 -- T17/RConn1
  B405/RConn2 -- L-35-2/RConn2 -- L-35-1/RConn2 -- T17/RConn2
  B405/RConn3 -- L-35-2/RConn3 -- L-35-1/RConn3 -- T17/RConn3
  B407/LConn1 -- Load20/LConn1 -- L-39/LConn1 -- T16/RConn1
  B407/LConn2 -- Load20/LConn2 -- L-39/LConn2 -- T16/RConn2
  B407/LConn3 -- Load20/LConn3 -- L-39/LConn3 -- T16/RConn3
  T15/RConn1 -- B408/RConn1 -- L-39/RConn1 -- L-36-1/RConn1
  B408/RConn2 -- L-39/RConn2 -- L-36-1/RConn2 -- T15/RConn2
  B408/RConn3 -- L-39/RConn3 -- L-36-1/RConn3 -- T15/RConn3
  B405/LConn1 -- L-36-1/LConn1 -- T405/RConn1 -- Load18/LConn1 -- L-37-2/LConn1 -- L-37-3/LConn1 -- L-37-1/LConn1
  B405/LConn2 -- T405/RConn2 -- Load18/LConn2 -- L-37-2/LConn2 -- L-37-3/LConn2 -- L-36-1/LConn2 -- L-37-1/LConn2
  T405/RConn3 -- Load18/LConn3 -- L-37-2/LConn3 -- L-37-3/LConn3 -- L-36-1/LConn3 -- B405/LConn3 -- L-37-1/LConn3
  L-37-2/RConn1 -- L-37-1/RConn1 -- B409/RConn1 -- L-37-3/RConn1
  L-37-2/RConn2 -- L-37-1/RConn2 -- B409/RConn2 -- L-37-3/RConn2
  B409/RConn3 -- L-37-2/RConn3 -- L-37-3/RConn3 -- L-37-1/RConn3
  B409/LConn1 -- Load22/LConn1 -- Comp4-409/LConn1 -- L-41-2/LConn1 -- L-41-1/LConn1
  B409/LConn2 -- Comp4-409/LConn2 -- Load22/LConn2 -- L-41-2/LConn2 -- L-41-1/LConn2
  B409/LConn3 -- Comp4-409/LConn3 -- Load22/LConn3 -- L-41-2/LConn3 -- L-41-1/LConn3
  B408/LConn1 -- Load21/LConn1 -- L-40-2/LConn1 -- L-40-1/LConn1
  Load21/LConn2 -- L-40-2/LConn2 -- B408/LConn2 -- L-40-1/LConn2
  B408/LConn3 -- Load21/LConn3 -- L-40-2/LConn3 -- L-40-1/LConn3
  B411/RConn1 -- L-42/RConn1 -- L-41-2/RConn1 -- L-41-1/RConn1 -- T36/RConn1
  L-41-2/RConn2 -- L-41-1/RConn2 -- T36/RConn2 -- L-42/RConn2 -- B411/RConn2
  B411/RConn3 -- L-42/RConn3 -- T36/RConn3 -- L-41-2/RConn3 -- L-41-1/RConn3
  T14/RConn1 -- L-40-1/RConn1 -- L-40-2/RConn1 -- B410/RConn1
  B410/RConn2 -- L-40-2/RConn2 -- L-40-1/RConn2 -- T14/RConn2
  T14/RConn3 -- L-40-2/RConn3 -- L-40-1/RConn3 -- B410/RConn3
  VI410_form/RConn1 -- B410_vi/LConn1 -- VI410/RConn1
  VI410_form/RConn2 -- B410_vi/LConn2 -- VI410/RConn2
  L-44-1/LConn3 -- T410/RConn3 -- L-43-3/LConn3 -- T35/RConn3 -- L-42/LConn3 -- Load23/LConn3 -- L-43-4/LConn3 -- B410/LConn3 -- L-43-2/LConn3 -- L-43-1/LConn3 -- L-44-2/LConn3
  B413/RConn1 -- L-44-2/RConn1 -- L-44-1/RConn1
  B413/RConn2 -- L-44-2/RConn2 -- L-44-1/RConn2
  B413/RConn3 -- L-44-2/RConn3 -- L-44-1/RConn3
  B411/LConn1 -- Comp5-411/LConn1 -- Load24/LConn1 -- L-45-2/LConn1 -- L-45-1/LConn1
  B411/LConn2 -- Comp5-411/LConn2 -- Load24/LConn2 -- L-45-2/LConn2 -- L-45-1/LConn2
  B411/LConn3 -- Comp5-411/LConn3 -- Load24/LConn3 -- L-45-2/LConn3 -- L-45-1/LConn3
  B412/RConn1 -- L-45-2/RConn1 -- L-45-1/RConn1 -- L-43-4/RConn1 -- L-43-3/RConn1 -- L-43-1/RConn1 -- L-43-2/RConn1
  B412/RConn2 -- L-45-2/RConn2 -- L-45-1/RConn2 -- L-43-4/RConn2 -- L-43-3/RConn2 -- L-43-1/RConn2 -- L-43-2/RConn2
  L-43-3/RConn3 -- L-43-1/RConn3 -- L-43-2/RConn3 -- L-45-2/RConn3 -- L-45-1/RConn3 -- L-43-4/RConn3 -- B412/RConn3
  Load25/LConn1 -- B412/LConn1
  Load25/LConn2 -- B412/LConn2
  Load25/LConn3 -- B412/LConn3
  B404/LConn3 -- T17/LConn3
  B404/LConn2 -- T17/LConn2
  B404/LConn1 -- T17/LConn1
  Load Flow Bus2/LConn1 -- B404/RConn3 -- G404_GPS/LConn3
  B403/RConn2 -- T16/LConn2
  B403/RConn1 -- T16/LConn1
  B403/RConn3 -- T16/LConn3
  CPS403/LConn3 -- B403/LConn3 -- Load Flow Bus15/LConn1 -- B403_vi/RConn3
  B402/RConn2 -- T15/LConn2
  Load Flow Bus3/LConn1 -- B402/LConn1 -- CPS402/LConn1
  B402/RConn3 -- T15/LConn3
  B402/RConn1 -- T15/LConn1
  B401/RConn2 -- T14/LConn2
  B401/RConn3 -- T14/LConn3
  B401/RConn1 -- T14/LConn1
  G401_TPS/LConn1 -- B401/LConn1 -- Load Flow Bus4/LConn1
  G401_TPS/LConn2 -- B401/LConn2
  G401_TPS/LConn3 -- B401/LConn3
  B413/LConn1 -- T18-2/LConn1 -- T18-1/LConn1
  B413/LConn2 -- T18-2/LConn2 -- T18-1/LConn2
  B413/LConn3 -- T18-2/LConn3 -- T18-1/LConn3
  B414/RConn2 -- T18-2/RConn2 -- T18-1/RConn2
  B414/RConn1 -- T18-2/RConn1 -- T18-1/RConn1
  B414/RConn3 -- T18-2/RConn3 -- T18-1/RConn3
  B415/RConn1 -- L-46-2/RConn1 -- L-46-1/RConn1
  B415/RConn2 -- L-46-2/RConn2 -- L-46-1/RConn2
  B415/RConn3 -- L-46-2/RConn3 -- L-46-1/RConn3
  B414/LConn1 -- Comp6-414/LConn1 -- L-46-2/LConn1 -- L-46-1/LConn1
  Comp6-414/LConn2 -- B414/LConn2 -- L-46-1/LConn2 -- L-46-2/LConn2
  B414/LConn3 -- Comp6-414/LConn3 -- L-46-2/LConn3 -- L-46-1/LConn3
  L-6-1/RConn1 -- Three-Phase V-I Measurement1/LConn1 -- L-6-2/RConn1
  L-6-1/RConn2 -- L-6-2/RConn2 -- Three-Phase V-I Measurement1/LConn2
  L-6-1/RConn3 -- L-6-2/RConn3 -- Three-Phase V-I Measurement1/LConn3
  B416/LConn1 -- Comp8-416/LConn1 -- L-6-2/LConn1 -- L-6-1/LConn1
  B416/LConn2 -- Comp8-416/LConn2 -- L-6-2/LConn2 -- L-6-1/LConn2
  B416/LConn3 -- Comp8-416/LConn3 -- L-6-2/LConn3 -- L-6-1/LConn3
  L-7-1/RConn1 -- T37/RConn1 -- B206/RConn1 -- L-5-1/RConn1 -- L-5-2/RConn1 -- T2/RConn1 -- L-7-2/RConn1
  B206/RConn2 -- T37/RConn2 -- L-7-1/RConn2 -- L-7-2/RConn2 -- T2/RConn2 -- L-5-2/RConn2 -- L-5-1/RConn2
  T2/RConn3 -- L-7-1/RConn3 -- L-7-2/RConn3 -- T37/RConn3 -- L-5-2/RConn3 -- L-5-1/RConn3 -- B206/RConn3
  Load2/LConn1 -- L-5-1/LConn1 -- B205/LConn1 -- L-5-2/LConn1
  Load2/LConn2 -- L-5-1/LConn2 -- B205/LConn2 -- L-5-2/LConn2
  Load2/LConn3 -- L-5-1/LConn3 -- L-5-2/LConn3 -- B205/LConn3
  G201_BPS/LConn1 -- B201/RConn1
  B201/LConn1 -- T2/LConn1
  G201_BPS/LConn3 -- Load Flow Bus6/LConn1 -- B201/RConn3
  B201/LConn2 -- T2/LConn2
  B201/LConn3 -- T2/LConn3
  G201_BPS/LConn2 -- B201/RConn2
  B207/LConn1 -- L-11/LConn1 -- L-7-2/LConn1 -- L-7-1/LConn1
  B207/LConn2 -- L-11/LConn2 -- L-7-2/LConn2 -- L-7-1/LConn2
  B207/LConn3 -- L-11/LConn3 -- L-7-2/LConn3 -- L-7-1/LConn3
  B207/RConn1 -- L-10-2/RConn1 -- L-10-1/RConn1 -- Load4/LConn1
  B207/RConn2 -- L-10-2/RConn2 -- L-10-1/RConn2 -- Load4/LConn2
  B207/RConn3 -- L-10-2/RConn3 -- L-10-1/RConn3 -- Load4/LConn3
  T4/RConn1 -- T208/RConn1 -- B208/RConn1 -- L-10-1/LConn1 -- L-10-2/LConn1
  VI208_form/RConn2 -- B208_vi/RConn2 -- VI208/RConn2
  T4/RConn3 -- T208/RConn3 -- B208/RConn3 -- L-10-1/LConn3 -- L-10-2/LConn3
  G203_VPS/LConn1 -- B203/RConn1
  B203/LConn1 -- T4/LConn1
  B203/LConn3 -- T4/LConn3
  G203_VPS/LConn2 -- B203/RConn2
  G203_VPS/LConn3 -- Load Flow Bus5/LConn1 -- B203/RConn3
  B203/LConn2 -- T4/LConn2
  L-12-3/LConn1 -- L-12-2/LConn1 -- L-12-1/LConn1 -- B211/RConn1
  L-12-3/LConn2 -- L-12-2/LConn2 -- L-12-1/LConn2 -- B211/RConn2
  L-12-3/LConn3 -- L-12-2/LConn3 -- B211/RConn3 -- L-12-1/LConn3
  Load5/LConn1 -- L-12-3/RConn1 -- L-12-2/RConn1 -- L-12-1/RConn1 -- B208/LConn1
  Load5/LConn2 -- L-12-3/RConn2 -- L-12-1/RConn2 -- B208/LConn2 -- L-12-2/RConn2
  Load5/LConn3 -- L-12-3/RConn3 -- L-12-2/RConn3 -- L-12-1/RConn3 -- B208/LConn3
  B211/LConn1 -- Load6/LConn1 -- L-16/RConn1 -- L-15-2/RConn1 -- L-15-1/RConn1
  L-16/RConn2 -- Load6/LConn2 -- L-15-2/RConn2 -- L-15-1/RConn2 -- B211/LConn2
  B211/LConn3 -- Load6/LConn3 -- L-16/RConn3 -- L-15-2/RConn3 -- L-15-1/RConn3
  B206/LConn1 -- L-9-1/RConn1 -- L-9-2/RConn1 -- Load3/LConn1 -- L-8-2/RConn1 -- L-8-1/RConn1
  L-9-1/RConn2 -- Load3/LConn2 -- L-8-2/RConn2 -- L-8-1/RConn2 -- B206/LConn2 -- L-9-2/RConn2
  B206/LConn3 -- L-9-1/RConn3 -- L-9-2/RConn3 -- Load3/LConn3 -- L-8-2/RConn3 -- L-8-1/RConn3
  L-15-2/LConn1 -- L-15-1/LConn1 -- T38/RConn1 -- L-8-1/LConn1 -- L-13/LConn1 -- B212/RConn1 -- L-8-2/LConn1
  B212/RConn2 -- L-13/LConn2 -- L-8-2/LConn2 -- T38/RConn2 -- L-15-2/LConn2 -- L-15-1/LConn2 -- L-8-1/LConn2
  L-15-2/LConn3 -- L-15-1/LConn3 -- T38/RConn3 -- L-8-2/LConn3 -- L-8-1/LConn3 -- L-13/LConn3 -- B212/RConn3
  T3/RConn3 -- L-11/RConn3 -- B209/RConn3
  T3/RConn2 -- L-11/RConn2 -- B209/RConn2
  T3/RConn1 -- L-11/RConn1 -- B209/RConn1
  B202/LConn2 -- T3/LConn2
  G202_EPS/LConn3 -- B202/RConn3
  B202/LConn3 -- T3/LConn3
  G202_EPS/LConn1 -- Load Flow Bus7/LConn1 -- B202/RConn1
  B202/LConn1 -- T3/LConn1
  G202_EPS/LConn2 -- B202/RConn2
  T6/LConn1 -- L-13/RConn1 -- B209/LConn1
  T6/LConn2 -- L-13/RConn2 -- B209/LConn2
  T6/LConn3 -- L-13/RConn3 -- B209/LConn3
  B210/RConn1 -- T6/RConn1
  B210/RConn2 -- T6/RConn2
  B210/RConn3 -- T6/RConn3
  B213/RConn1 -- L-14-1/LConn1 -- L-14-2/LConn1
  B213/RConn2 -- L-14-1/LConn2 -- L-14-2/LConn2
  B213/RConn3 -- L-14-1/LConn3 -- L-14-2/LConn3
  B210/LConn1 -- L-14-2/RConn1 -- L-14-1/RConn1
  B210/LConn2 -- L-14-2/RConn2 -- L-14-1/RConn2
  B210/LConn3 -- L-14-2/RConn3 -- L-14-1/RConn3
  L-17/RConn1 -- T212/RConn1 -- Comp2-212/LConn1 -- Load7/LConn1 -- B212/LConn1
  B212/LConn2 -- Load7/LConn2 -- T212/RConn2 -- Comp2-212/LConn2 -- L-17/RConn2
  B212/LConn3 -- Load7/LConn3 -- T212/RConn3 -- Comp2-212/LConn3 -- L-17/RConn3
  B214/RConn2 -- L-16/LConn2 -- T7/RConn2
  B214/RConn1 -- L-16/LConn1 -- T7/RConn1
  B214/RConn3 -- L-16/LConn3 -- T7/RConn3
  T7/LConn1 -- B213/LConn1
  T7/LConn2 -- B213/LConn2
  T7/LConn3 -- B213/LConn3
  L-18/LConn2 -- T216/RConn2 -- L-20-1/LConn2 -- L-20-2/LConn2 -- B216/RConn2
  L-18/LConn1 -- T216/RConn1 -- L-20-1/LConn1 -- L-20-2/LConn1 -- B216/RConn1
  L-18/LConn3 -- B216/RConn3 -- T216/RConn3 -- L-20-1/LConn3 -- L-20-2/LConn3
  B214/LConn3 -- L-19/RConn3 -- L-18/RConn3
  B214/LConn1 -- L-19/RConn1 -- L-18/RConn1
  B214/LConn2 -- L-19/RConn2 -- L-18/RConn2
  L-22/LConn1 -- L-19/LConn1 -- L-17/LConn1 -- L-21-2/LConn1 -- L-21-1/LConn1 -- B217/RConn1
  L-22/LConn2 -- L-19/LConn2 -- L-17/LConn2 -- L-21-1/LConn2 -- L-21-2/LConn2 -- B217/RConn2
  L-22/LConn3 -- L-19/LConn3 -- L-17/LConn3 -- L-21-1/LConn3 -- L-21-2/LConn3 -- B217/RConn3
  L-22/RConn1 -- Comp3-216/LConn1 -- Load9/LConn1 -- B216/LConn1
  L-22/RConn2 -- Comp3-216/LConn2 -- Load9/LConn2 -- B216/LConn2
  L-22/RConn3 -- Comp3-216/LConn3 -- Load9/LConn3 -- B216/LConn3
  B215/RConn1 -- L-9-2/LConn1 -- L-9-1/LConn1
  B215/RConn2 -- L-9-2/LConn2 -- L-9-1/LConn2
  B215/RConn3 -- L-9-2/LConn3 -- L-9-1/LConn3
  T5/RConn1 -- Load8/LConn1 -- T215/RConn1 -- L-21-2/RConn1 -- L-21-1/RConn1 -- L-20-2/RConn1 -- L-20-1/RConn1 -- B215/LConn1
  T5/RConn2 -- Load8/LConn2 -- T215/RConn2 -- L-21-2/RConn2 -- L-21-1/RConn2 -- L-20-2/RConn2 -- L-20-1/RConn2 -- B215/LConn2
  T5/RConn3 -- Load8/LConn3 -- T215/RConn3 -- L-21-2/RConn3 -- L-21-1/RConn3 -- L-20-2/RConn3 -- L-20-1/RConn3 -- B215/LConn3
  L-2-1/RConn1 -- L-1-1/RConn1 -- L-1-2/RConn1 -- L-2-2/RConn1 -- Three-Phase V-I Measurement2/LConn1
  L-2-2/RConn3 -- Three-Phase V-I Measurement2/LConn3 -- L-1-1/RConn3 -- L-1-2/RConn3 -- L-2-1/RConn3
  L-1-1/LConn1 -- B217/LConn1 -- Load10/LConn1 -- L-2-2/LConn1 -- L-2-1/LConn1 -- L-1-2/LConn1
  B217/LConn2 -- Load10/LConn2 -- L-2-2/LConn2 -- L-2-1/LConn2 -- L-1-2/LConn2 -- L-1-1/LConn2
  L-1-1/LConn3 -- Load10/LConn3 -- L-2-2/LConn3 -- L-2-1/LConn3 -- L-1-2/LConn3 -- B217/LConn3
  L-3-1/RConn1 -- L-4/RConn1 -- L-3-2/RConn1 -- Three-Phase V-I Measurement3/LConn1
  L-3-1/RConn2 -- L-4/RConn2 -- L-3-2/RConn2 -- Three-Phase V-I Measurement3/LConn2
  L-3-1/RConn3 -- L-4/RConn3 -- L-3-2/RConn3 -- Three-Phase V-I Measurement3/LConn3
  B102/LConn1 -- L-3-1/LConn1 -- T1/RConn1 -- Load1/LConn1 -- L-4/LConn1 -- L-3-2/LConn1
  B102/LConn2 -- L-3-1/LConn2 -- T1/RConn2 -- Load1/LConn2 -- L-4/LConn2 -- L-3-2/LConn2
  B102/LConn3 -- L-3-1/LConn3 -- T1/RConn3 -- Load1/LConn3 -- L-4/LConn3 -- L-3-2/LConn3
  B101/LConn1 -- T1/LConn1
  Load Flow Bus9/LConn1 -- 3-Phase Dynamic Load4/LConn3 -- B101/RConn3
  B101/LConn3 -- T1/LConn3
  B101/LConn2 -- T1/LConn2
  L-30-2/LConn2 -- B309/LConn2 -- Load14/LConn2 -- L-30-1/LConn2
  L-30-2/LConn3 -- B309/LConn3 -- Load14/LConn3 -- L-30-1/LConn3
  T11/LConn1 -- T12/LConn1 -- B305/RConn1 -- L-24-1/LConn1 -- L-24-2/LConn1 -- L-25/LConn1
  T11/LConn2 -- T12/LConn2 -- B305/RConn2 -- L-24-1/LConn2 -- L-24-2/LConn2 -- L-25/LConn2
  T11/LConn3 -- T12/LConn3 -- B305/RConn3 -- L-24-1/LConn3 -- L-24-2/LConn3 -- L-25/LConn3
  L-24-2/RConn1 -- L-24-1/RConn1 -- L-23/RConn1 -- B303/RConn1
  L-24-2/RConn2 -- L-24-1/RConn2 -- L-23/RConn2 -- B303/RConn2
  L-24-2/RConn3 -- L-24-1/RConn3 -- L-23/RConn3 -- B303/RConn3
  B307/RConn1 -- L-28/LConn1 -- T39/RConn1 -- L-27-2/LConn1 -- L-27-1/LConn1
  B307/RConn2 -- L-28/LConn2 -- T39/RConn2 -- L-27-2/LConn2 -- L-27-1/LConn2
  B307/RConn3 -- L-28/LConn3 -- T39/RConn3 -- L-27-2/LConn3 -- L-27-1/LConn3
  B305/LConn1 -- L-26/RConn1 -- L-27-2/RConn1 -- L-27-1/RConn1
  B305/LConn2 -- L-26/RConn2 -- L-27-2/RConn2 -- L-27-1/RConn2
  B305/LConn3 -- L-26/RConn3 -- L-27-2/RConn3 -- L-27-1/RConn3
  L-25/RConn1 -- B304/LConn1
  L-25/RConn2 -- B304/LConn2
  L-25/RConn3 -- B304/LConn3
  G301_LPS/LConn2 -- B301/LConn2
  G301_LPS/LConn1 -- B301/LConn1
  G301_LPS/LConn3 -- Load Flow Bus10/LConn1 -- B301/LConn3
  T8/LConn1 -- B301/RConn1
  T8/LConn3 -- B301/RConn3
  T8/LConn2 -- B301/RConn2
  T8/RConn1 -- B303/LConn1
  T8/RConn2 -- B303/LConn2
  T8/RConn3 -- B303/LConn3
  B304/RConn1 -- L-23/LConn1 -- T10/LConn1
  B304/RConn2 -- L-23/LConn2 -- T10/LConn2
  T10/LConn3 -- L-23/LConn3 -- B304/RConn3
  L-33/LConn1 -- B314/RConn1
  L-33/LConn2 -- B314/RConn2
  L-33/LConn3 -- B314/RConn3
  L-33/RConn1 -- B313/LConn1
  L-33/RConn2 -- B313/LConn2
  L-33/RConn3 -- B313/LConn3
  T12/RConn3 -- Load17/LConn3 -- T314/RConn3 -- B314/LConn3
  T12/RConn2 -- T314/RConn2 -- Load17/LConn2 -- B314/LConn2
  T12/RConn1 -- T314/RConn1 -- Load17/LConn1 -- B314/LConn1
  T10/RConn1 -- B313/RConn1 -- Load16/LConn1 -- L-32/LConn1
  B313/RConn2 -- Load16/LConn2 -- L-32/LConn2 -- T10/RConn2
  T10/RConn3 -- B313/RConn3 -- Load16/LConn3 -- L-32/LConn3
  B312/LConn2 -- Load15/LConn2 -- L-32/RConn2
  L-32/RConn1 -- Load15/LConn1 -- B312/LConn1
  L-32/RConn3 -- Load15/LConn3 -- B312/LConn3
  G302_YPS/LConn3 -- B302/LConn3 -- Load Flow Bus11/LConn1
  T9/LConn3 -- B302/RConn3
  B312/RConn3 -- T312/RConn3 -- T9/RConn3
  T9/LConn2 -- B302/RConn2
  T9/LConn1 -- B302/RConn1
  B312/RConn2 -- T312/RConn2 -- T9/RConn2
  G302_YPS/LConn1 -- B302/LConn1
  G302_YPS/LConn2 -- B302/LConn2
  B312/RConn1 -- T312/RConn1 -- T9/RConn1
  B306/RConn1 -- L-26/LConn1 -- Load11/LConn1
  L-26/LConn2 -- Load11/LConn2 -- B306/RConn2
  B306/RConn3 -- L-26/LConn3 -- Load11/LConn3
  L-28/RConn1 -- B306/LConn1
  L-28/RConn2 -- B306/LConn2
  L-28/RConn3 -- B306/LConn3
  T11/RConn1 -- B311/LConn1
  T11/RConn2 -- B311/LConn2
  T11/RConn3 -- B311/LConn3
  B308/LConn1 -- Load13/LConn1 -- T13/LConn1
  B308/LConn2 -- Load13/LConn2 -- T13/LConn2
  B308/LConn3 -- Load13/LConn3 -- T13/LConn3
  T13/RConn1 -- B315/LConn1
  T13/RConn2 -- B315/LConn2
  T13/RConn3 -- B315/LConn3
  L-49-2/LConn1 -- B504/LConn1 -- L-48-1/LConn1 -- L-48-2/LConn1 -- L-49-1/LConn1
  L-49-2/LConn2 -- L-49-1/LConn2 -- L-48-1/LConn2 -- B504/LConn2 -- L-48-2/LConn2
  L-49-2/LConn3 -- L-49-1/LConn3 -- B504/LConn3 -- L-48-1/LConn3 -- L-48-2/LConn3
  B507/RConn2 -- Load27/LConn2 -- L-50-1/LConn2 -- L-48-2/RConn2 -- L-48-1/RConn2
  B507/RConn1 -- Load27/LConn1 -- L-48-2/RConn1 -- L-48-1/RConn1 -- L-50-1/LConn1
  B507/RConn3 -- Load27/LConn3 -- L-48-2/RConn3 -- L-48-1/RConn3 -- L-50-1/LConn3
  B509/RConn1 -- L-55-2/RConn1 -- L-55-1/RConn1
  B509/RConn2 -- L-55-2/RConn2 -- L-55-1/RConn2
  B509/RConn3 -- L-55-2/RConn3 -- L-55-1/RConn3
  L-55-2/LConn1 -- L-54/LConn1 -- L-55-1/LConn1 -- L-52/LConn1 -- B507/LConn1
  B507/LConn2 -- L-55-1/LConn2 -- L-52/LConn2 -- L-54/LConn2 -- L-55-2/LConn2
  L-54/LConn3 -- L-55-2/LConn3 -- B507/LConn3 -- L-55-1/LConn3 -- L-52/LConn3
  B509/LConn1 -- Load29/LConn1 -- L-34-1/LConn1 -- L-34-2/LConn1
  Load29/LConn2 -- L-34-2/LConn2 -- L-34-1/LConn2 -- B509/LConn2
  B509/LConn3 -- L-34-1/LConn3 -- Load29/LConn3 -- L-34-2/LConn3
  G503_PPS/LConn3 -- B503/LConn3 -- Load Flow Bus12/LConn1
  G503_PPS/LConn1 -- B503/LConn1
  G503_PPS/LConn2 -- B503/LConn2
  B506/RConn1 -- L-53/RConn1 -- L-52/RConn1
  B506/RConn2 -- L-53/RConn2 -- L-52/RConn2
  B506/RConn3 -- L-53/RConn3 -- L-52/RConn3
  B506/LConn2 -- T21/RConn2
  B506/LConn3 -- T21/RConn3
  B506/LConn1 -- T21/RConn1
  L-49-2/RConn1 -- L-49-1/RConn1 -- L-51/RConn1 -- L-54/RConn1 -- L-53/LConn1 -- B508/RConn1
  L-49-2/RConn2 -- L-49-1/RConn2 -- L-51/RConn2 -- L-54/RConn2 -- L-53/LConn2 -- B508/RConn2
  L-49-2/RConn3 -- L-49-1/RConn3 -- L-51/RConn3 -- L-54/RConn3 -- L-53/LConn3 -- B508/RConn3
  Load28/LConn1 -- T40/RConn1 -- T508/RConn1 -- B508/LConn1
  Load28/LConn2 -- T508/RConn2 -- T40/RConn2 -- B508/LConn2
  Load28/LConn3 -- T40/RConn3 -- T508/RConn3 -- B508/LConn3
  B505/RConn1 -- L-51/LConn1 -- L-50-1/RConn1
  B505/RConn2 -- L-51/LConn2 -- L-50-1/RConn2
  B505/RConn3 -- L-51/LConn3 -- L-50-1/RConn3
  B505/LConn3 -- T502/RConn3 -- T20/RConn3
  B502/RConn2 -- T20/LConn2
  B502/RConn1 -- T20/LConn1
  B505/LConn2 -- T502/RConn2 -- T20/RConn2
  B502/RConn3 -- T20/LConn3
  B505/LConn1 -- T502/RConn1 -- T20/RConn1
  B501/LConn2 -- T19/LConn2
  B501/LConn3 -- T19/LConn3
  B501/LConn1 -- T19/LConn1
  B504/RConn2 -- Load26/LConn2 -- T504/RConn2 -- T19/RConn2
  B504/RConn1 -- Load26/LConn1 -- T504/RConn1 -- T19/RConn1
  B504/RConn3 -- Load26/LConn3 -- T19/RConn3 -- T504/RConn3
  Load19/LConn1 -- B406/LConn1
  Load19/LConn2 -- B406/LConn2
  Load19/LConn3 -- B406/LConn3
  B204/LConn3 -- T5/LConn3
  G204_MPS/LConn1 -- Load Flow Bus8/LConn1 -- B204/RConn1
  G204_MPS/LConn3 -- B204/RConn3
  G204_MPS/LConn2 -- B204/RConn2
  B204/LConn1 -- T5/LConn1
  B204/LConn2 -- T5/LConn2
  B415/LConn1 -- Comp7-415/LConn1 -- L-47-2/LConn1 -- L-47-1/LConn1
  B415/LConn2 -- Comp7-415/LConn2 -- L-47-2/LConn2 -- L-47-1/LConn2
  B415/LConn3 -- Comp7-415/LConn3 -- L-47-2/LConn3 -- L-47-1/LConn3
  B416/RConn2 -- L-47-1/RConn2 -- L-47-2/RConn2
  B416/RConn3 -- L-47-1/RConn3 -- L-47-2/RConn3
  B416/RConn1 -- L-47-1/RConn1 -- L-47-2/RConn1
  B308/RConn1 -- T308/RConn1 -- L-29-1/LConn1 -- L-29-2/LConn1
  B308/RConn2 -- T308/RConn2 -- L-29-1/LConn2 -- L-29-2/LConn2
  B308/RConn3 -- T308/RConn3 -- L-29-1/LConn3 -- L-29-2/LConn3
  B307/LConn1 -- Load12/LConn1 -- L-29-1/RConn1 -- L-29-2/RConn1
  B307/LConn2 -- Load12/LConn2 -- L-29-1/RConn2 -- L-29-2/RConn2
  B307/LConn3 -- Load12/LConn3 -- L-29-1/RConn3 -- L-29-2/RConn3
  B205/RConn3 -- Three-Phase V-I Measurement1/RConn3
  B205/RConn2 -- Three-Phase V-I Measurement1/RConn2
  B205/RConn1 -- Three-Phase V-I Measurement1/RConn1
  L-30-2/LConn1 -- L-30-1/LConn1 -- B309/LConn1 -- Load14/LConn1
  2/RConn1 -- B310/LConn1 -- 1/RConn1
  1/RConn2 -- 2/RConn2 -- B310/LConn2
  2/RConn3 -- B310/LConn3 -- 1/RConn3
  2/LConn1 -- B311/RConn1 -- 1/LConn1
  2/LConn2 -- B311/RConn2 -- 1/LConn2
  1/LConn3 -- 2/LConn3 -- B311/RConn3
  L-2-1/RConn2 -- L-1-1/RConn2 -- L-1-2/RConn2 -- Three-Phase V-I Measurement2/LConn2 -- L-2-2/RConn2
  B102/RConn1 -- T102/RConn1 -- Three-Phase V-I Measurement2/RConn1
  B102/RConn2 -- T102/RConn2 -- Three-Phase V-I Measurement2/RConn2
  B102/RConn3 -- T102/RConn3 -- Three-Phase V-I Measurement2/RConn3
  L-30-1/RConn1 -- L-30-2/RConn1 -- B310/RConn1
  L-30-1/RConn2 -- L-30-2/RConn2 -- B310/RConn2
  L-30-1/RConn3 -- L-30-2/RConn3 -- B310/RConn3
  Three-Phase V-I Measurement3/RConn1 -- T309/RConn1 -- B309/RConn1
  Three-Phase V-I Measurement3/RConn2 -- T309/RConn2 -- B309/RConn2
  Three-Phase V-I Measurement3/RConn3 -- T309/RConn3 -- B309/RConn3
  B315/RConn3 -- Three-Phase V-I Measurement4/LConn3
  B315/RConn2 -- Three-Phase V-I Measurement4/LConn2
  B315/RConn1 -- Three-Phase V-I Measurement4/LConn1
  G404_GPS/LConn2 -- B404/RConn2
  G404_GPS/LConn1 -- B404/RConn1
  CPS403/LConn2 -- B403_vi/RConn2 -- B403/LConn2
  CPS403/LConn1 -- B403/LConn1 -- B403_vi/RConn1
  B402/LConn2 -- CPS402/LConn2
  CPS402/LConn3 -- B402/LConn3
  Load Flow Bus13/LConn1 -- 3-Phase Dynamic Load3/LConn3 -- B502/LConn3
  G501_NPS/LConn1 -- B501/RConn1
  B501/RConn2 -- G501_NPS/LConn2
  G501_NPS/LConn3 -- Load Flow Bus14/LConn1 -- B501/RConn3
  B312_vi/LConn3 -- T312/LConn3
  T312/LConn2 -- B312_vi/LConn2
  T312/LConn1 -- B312_vi/LConn1
  B314_vi/LConn3 -- T314/LConn3
  T314/LConn1 -- B314_vi/LConn1
  T314/LConn2 -- B314_vi/LConn2
  T308/LConn2 -- B308_vi/RConn2
  T308/LConn3 -- B308_vi/RConn3
  T308/LConn1 -- B308_vi/RConn1
  T504/LConn3 -- B504_vi/RConn3
  T504/LConn1 -- B504_vi/RConn1
  T504/LConn2 -- B504_vi/RConn2
  B508_vi/RConn3 -- T508/LConn1
  T508/LConn2 -- B508_vi/RConn2
  B508_vi/RConn1 -- T508/LConn3
  T309/LConn1 -- B309_vi/LConn3
  T309/LConn2 -- B309_vi/LConn2
  T309/LConn3 -- B309_vi/LConn1
  B102_vi/LConn1 -- T102/LConn1
  B102_vi/LConn2 -- T102/LConn2
  B102_vi/LConn3 -- T102/LConn3
  T216/LConn1 -- B216_vi/RConn1
  T216/LConn2 -- B216_vi/RConn2
  T216/LConn3 -- B216_vi/RConn3
  T502/LConn1 -- B502_vi/RConn1
  T502/LConn2 -- B502_vi/RConn2
  T502/LConn3 -- B502_vi/RConn3
  Dist410/RConn1 -- T35/LConn1
  Dist410/RConn2 -- T35/LConn2
  Dist410/RConn3 -- T35/LConn3
  T36/LConn1 -- Dist411/RConn1
  T36/LConn2 -- Dist411/RConn2
  T36/LConn3 -- Dist411/RConn3
  T37/LConn1 -- Dist206/RConn1
  T37/LConn3 -- Dist206/RConn3
  T37/LConn2 -- Dist206/RConn2
  T38/LConn1 -- Dist212/RConn1
  T38/LConn2 -- Dist212/RConn2
  T38/LConn3 -- Dist212/RConn3
  T39/LConn1 -- Dist307/RConn1
  T39/LConn2 -- Dist307/RConn2
  T39/LConn3 -- Dist307/RConn3
  T40/LConn1 -- Dist508/RConn1
  T40/LConn2 -- Dist508/RConn2
  T40/LConn3 -- Dist508/RConn3
  3-Phase Dynamic Load3/LConn1 -- B502/LConn1
  B502/LConn2 -- 3-Phase Dynamic Load3/LConn2
  3-Phase Dynamic Load4/LConn1 -- B101/RConn1
  3-Phase Dynamic Load4/LConn2 -- B101/RConn2
  L-34-2/RConn2 -- Three-Phase Breaker/RConn2 -- L-34-1/RConn2
  L-34-2/RConn1 -- Three-Phase Breaker/RConn1 -- L-34-1/RConn1
  L-34-2/RConn3 -- Three-Phase Breaker/RConn3 -- L-34-1/RConn3
  Three-Phase Breaker2/LConn2 -- B503/RConn2 -- Three-Phase Breaker1/LConn2
  Three-Phase Breaker1/RConn2 -- T21/LConn2
  Three-Phase Breaker1/RConn1 -- T21/LConn1
  Three-Phase Breaker1/RConn3 -- T21/LConn3
  Three-Phase Breaker1/LConn1 -- B503/RConn1 -- Three-Phase Breaker2/LConn1
  Load30/LConn1 -- Three-Phase Breaker2/RConn1
  Load30/LConn2 -- Three-Phase Breaker2/RConn2
  Load30/LConn3 -- Three-Phase Breaker2/RConn3
  B503/RConn3 -- Three-Phase Breaker2/LConn3 -- Three-Phase Breaker1/LConn3
  Three-Phase Breaker/LConn3 -- Three-Phase V-I Measurement4/RConn3
  Three-Phase Breaker/LConn2 -- Three-Phase V-I Measurement4/RConn2
  Three-Phase Breaker/LConn1 -- Three-Phase V-I Measurement4/RConn1
  VI216_form/LConn1 -- VI216/RConn1 -- B216_vi/LConn1
  VI216_form/LConn2 -- VI216/RConn2 -- B216_vi/LConn2
  VI216_form/LConn3 -- VI216/RConn3 -- B216_vi/LConn3
  VI403_form/RConn1 -- B403_vi/LConn1 -- VI403/RConn1
  VI403_form/RConn2 -- B403_vi/LConn2 -- VI403/RConn2
  VI403_form/RConn3 -- B403_vi/LConn3 -- VI403/RConn3
  VI102_form/RConn1 -- VI102/RConn1 -- B102_vi/RConn1
  VI102_form/RConn2 -- VI102/RConn2 -- B102_vi/RConn2
  VI102_form/RConn3 -- VI102/RConn3 -- B102_vi/RConn3
  B212_vi/LConn1 -- T212/LConn1
  VI212_form/RConn1 -- VI212/RConn1 -- B212_vi/RConn1
  T212/LConn2 -- B212_vi/LConn2
  VI212_form/RConn3 -- VI212/RConn3 -- B212_vi/RConn3
  B212_vi/LConn3 -- T212/LConn3
  VI212_form/RConn2 -- VI212/RConn2 -- B212_vi/RConn2
  T208/LConn1 -- B208_vi/LConn1
  T208/LConn2 -- B208_vi/LConn2
  T208/LConn3 -- B208_vi/LConn3
  VI208_form/RConn3 -- B208_vi/RConn3 -- VI208/RConn3
  L-10-1/LConn2 -- T208/RConn2 -- B208/RConn2 -- T4/RConn2 -- L-10-2/LConn2
  B208_vi/RConn1 -- VI208/RConn1 -- VI208_form/RConn1
  T405/LConn2 -- B405_vi/LConn2
  T405/LConn1 -- B405_vi/LConn1
  T405/LConn3 -- B405_vi/LConn3
  B405_vi/RConn1 -- VI405/RConn1 -- VI405_form/RConn1
  B405_vi/RConn2 -- VI405/RConn2 -- VI405_form/RConn2
  B405_vi/RConn3 -- VI405/RConn3 -- VI405_form/RConn3
  VI410_form/RConn3 -- B410_vi/LConn3 -- VI410/RConn3
  Voltage Measurement/LConn2 -- T410/RConn1 -- L-44-1/LConn1 -- L-44-2/LConn1 -- L-43-1/LConn1 -- L-43-2/LConn1 -- L-43-3/LConn1 -- B410/LConn1 -- L-43-4/LConn1 -- T35/RConn1 -- L-42/LConn1 -- Load23/LConn1
  L-43-4/LConn2 -- T410/RConn2 -- L-44-1/LConn2 -- L-44-2/LConn2 -- L-43-1/LConn2 -- L-43-2/LConn2 -- L-43-3/LConn2 -- B410/LConn2 -- Load23/LConn2 -- Voltage Measurement/LConn1 -- L-42/LConn2 -- T35/RConn2
  T410/LConn3 -- B410_vi/RConn3
  T410/LConn1 -- B410_vi/RConn1
  T410/LConn2 -- B410_vi/RConn2
  VI309_form/RConn1 -- VI309/RConn1 -- B309_vi/RConn3
  VI309_form/RConn2 -- VI309/RConn2 -- B309_vi/RConn2
  VI309_form/RConn3 -- VI309/RConn3 -- B309_vi/RConn1
  VI312_form/LConn1 -- VI312/RConn1 -- B312_vi/RConn1
  VI312_form/LConn2 -- VI312/RConn2 -- B312_vi/RConn2
  VI312_form/LConn3 -- VI312/RConn3 -- B312_vi/RConn3
  VI314_form/LConn1 -- VI314/RConn1 -- B314_vi/RConn1
  VI314_form/LConn2 -- VI314/RConn2 -- B314_vi/RConn2
  VI314_form/LConn3 -- VI314/RConn3 -- B314_vi/RConn3
  VI308_form/LConn1 -- VI308/RConn1 -- B308_vi/LConn1
  VI308_form/LConn2 -- VI308/RConn2 -- B308_vi/LConn2
  VI308_form/LConn3 -- VI308/RConn3 -- B308_vi/LConn3
  B508_vi/LConn3 -- VI508/RConn1 -- VI508_form/LConn1
  B508_vi/LConn2 -- VI508/RConn2 -- VI508_form/LConn2
  B508_vi/LConn1 -- VI508/RConn3 -- VI508_form/LConn3
  VI504_form/LConn1 -- VI504/RConn1 -- B504_vi/LConn1
  VI504_form/LConn2 -- VI504/RConn2 -- B504_vi/LConn2
  VI504_form/LConn3 -- VI504/RConn3 -- B504_vi/LConn3
  VI502_form/LConn1 -- VI502/RConn1 -- B502_vi/LConn1
  VI502_form/LConn2 -- VI502/RConn2 -- B502_vi/LConn2
  VI502_form/LConn3 -- VI502/RConn3 -- B502_vi/LConn3
  VI215/RConn1 -- B215_vi/RConn3 -- VI215_form/LConn1
  VI215/RConn2 -- B215_vi/RConn2 -- VI215_form/LConn2
  VI215/RConn3 -- B215_vi/RConn1 -- VI215_form/LConn3
  T215/LConn1 -- B215_vi/LConn3
  T215/LConn2 -- B215_vi/LConn2
  T215/LConn3 -- B215_vi/LConn1
